simulink library "nist_library"  (R2012b)
settings: Solver=VariableStepDiscrete  StartTime=0  StopTime=1000  RelTol=1e-3
undefined symbols (not defined in the file or in its folder): A, B, C, D, sfp, xlipgetpartsetting
libraries: xbsIndex_r4 x385, xps_library x44, nist_library x4, casper_library_misc x4, casper_library_delays x1
(part 4 of 11)

== system nist_library/channelized_fir/odd_sym_tap ==
  samp_in : Inport
  sum_in : Inport  Port=2
  Constant0 : xbsIndex_r4/Constant  const=4  gui_display_data_type=Fixed-point  arith_type=Signed (2's comp)  n_bits=18  bin_pt=0  preci_type=Single  exp_width=8  frac_width=24  explicit_period=on  period=1  equ=P=C  opselect=C  inp2=PCIN>>17  opr=+  inp1=P  carry=CIN  dbl_ovrd=off  block_type=constant
  DSP48 Macro_0 : xbsIndex_r4/DSP48 Macro 2.1   dsptype=Target XtremeDSP Slice: DSP48E1  instruction_list=A * B+C  AvailableInstructions=|  show_filtered=off  pipeline_options=Expert  dspimage=|  tier_1=off  tier_2=off  tier_3=off  tier_4=off  tier_5=off  tier_6=off  dreg_1=off  dreg_2=off  dreg_3=off  areg_1=off  areg_2=off  areg_3=on  areg_4=on  breg_1=off  breg_2=off  breg_3=on  breg_4=on  mreg_5=on  concatreg_3=off  concatreg_4=off  concatreg_5=off  creg_1=off  creg_2=off  creg_3=off  creg_4=off  creg_5=on  preg_6=on  cinreg_1=off  cinreg_2=off  cinreg_3=off  cinreg_4=off  cinreg_5=off  opreg_1=off  opreg_2=off  opreg_3=off  opreg_4=off  opreg_5=off  output_properties=Full_Precision  p_width=39  p_binarywidth=0  has_acout=off  has_bcout=off  has_pcout=off  has_carryout=off  has_carrycascout=off  has_ce=off  has_d_ce=off  has_a_ce=off  has_b_ce=off  has_concat_ce=off  has_c_ce=off  has_m_ce=off  has_p_ce=off  has_sel_ce=off  has_sclr=off  has_d_sclr=off  has_a_sclr=off  has_b_sclr=off  has_concat_sclr=off  has_c_sclr=off  has_m_sclr=off  has_p_sclr=off  has_sel_sclr=off  use_dsp48=on  gui_behaviour=Sysgen  instruction1=#  ip_name=DSP48 Macro  ip_version=2.1  dsptool_ready=true  ipcore_usecache=true  ipcore_useipmodelcache=true  wrapper_available=true  port_translation_map={ 'ce' => 'en', 'sclr' => 'rst'}  ipcore_xco_need_fpga_part=true  ipcore_fpga_part=xlipgetpartsetting(gcb, {'virtex6', 'xc6vlx75t', '-3', 'ff784'})  ipcore_latency_function='has_combinational'  structural_sim=false  ipcore_verbose=false  ipcore_port_config={ 'carryin' => { 'arith' => 'ufix', 'binpt' => 0.00000000000, 'width' => 1.00000000000}, 'carrycascin' => { 'arith' => 'ufix', 'binpt' => 0.00000000000, 'width' => 1.00000000000}, 'carrycascout' => { 'arith' => 'ufix', 'binpt' => 0.00000000000, 'width' => 1.00000000000}, 'carryout' => { 'arith' => 'ufix', 'binpt' => 0.00000000000, 'width' => 1.00000000000}}  block_type=xbip_dsp48_macro_v2_1
      AvailableInstructions=|
      | '(A+D)
      | (A+D)*B
      | (A+D)*B+C
      | (A+D)*B+C+CARRYIN
      | (A+D)*B+CARRYIN
      | (A+D)*B+P
      | (A+D)*B+P+CARRYIN
      | (A+D)*B+P>>17
      | (A+D)*B+P>>17+CARRYIN
      | (A+D)*B+PCIN
      | (A+D)*B+PCIN+CARRYIN
      | (A+D)*B+PCIN>>17
      | (A+D)*B+PCIN>>17+CARRYIN
      | (A+D)*BCIN
      | (A+D)*BCIN+C
      | (A+D)*BCIN+C+CARRYIN
      | (A+D)*BCIN+CARRYIN
      | (A+D)*BCIN+P
      | (A+D)*BCIN+P+CARRYIN
      | (A+D)*BCIN+P>>17
      | (A+D)*BCIN+P>>17+CARRYIN
      | (A+D)*BCIN+PCIN
      | (A+D)*BCIN+PCIN+CARRYIN
      | (A+D)*BCIN+PCIN>>17
      | (A+D)*BCIN+PCIN>>17+CARRYIN
      | (A+D)+C
      | (A+D)+C+CARRYIN
      | (A+D)+CARRYIN
      | (A+D)+P
      | (A+D)+P+CARRYIN
      | (A+D)+P>>17
      | (A+D)+P>>17+CARRYIN
      | (A+D)+PCIN
      | (A+D)+PCIN+CARRYIN
      | (A+D)+PCIN>>17
      | (A+D)+PCIN>>17+CARRYIN
      | (ACIN+D)
      | (ACIN+D)*B
      | (ACIN+D)*B+C
      | (ACIN+D)*B+C+CARRYIN
      | (ACIN+D)*B+CARRYIN
      | (ACIN+D)*B+P
      | (ACIN+D)*B+P+CARRYIN
      | (ACIN+D)*B+P>>17
      | (ACIN+D)*B+P>>17+CARRYIN
      | (ACIN+D)*B+PCIN
      | (ACIN+D)*B+PCIN+CARRYIN
      | (ACIN+D)*B+PCIN>>17
      | (ACIN+D)*B+PCIN>>17+CARRYIN
      | (ACIN+D)*BCIN
      | (ACIN+D)*BCIN+C
      | (ACIN+D)*BCIN+C+CARRYIN
      | (ACIN+D)*BCIN+CARRYIN
      | (ACIN+D)*BCIN+P
      | (ACIN+D)*BCIN+P+CARRYIN
      | (ACIN+D)*BCIN+P>>17
      | (ACIN+D)*BCIN+P>>17+CARRYIN
      | (ACIN+D)*BCIN+PCIN
      | (ACIN+D)*BCIN+PCIN+CARRYIN
      | (ACIN+D)*BCIN+PCIN>>17
      | (ACIN+D)*BCIN+PCIN>>17+CARRYIN
      | (ACIN+D)+C
      | (ACIN+D)+C+CARRYIN
      | (ACIN+D)+CARRYIN
      | (ACIN+D)+P
      | (ACIN+D)+P+CARRYIN
      | (ACIN+D)+P>>17
      | (ACIN+D)+P>>17+CARRYIN
      | (ACIN+D)+PCIN
      | (ACIN+D)+PCIN+CARRYIN
      | (ACIN+D)+PCIN>>17
      | (ACIN+D)+PCIN>>17+CARRYIN
      | (D+A)
      | (D+A)*B
      | (D+A)*B+C
      | (D+A)*B+C+CARRYIN
      | (D+A)*B+CARRYIN
      | (D+A)*B+P
      | (D+A)*B+P+CARRYIN
      | (D+A)*B+P>>17
      | (D+A)*B+P>>17+CARRYIN
      | (D+A)*B+PCIN
      | (D+A)*B+PCIN+CARRYIN
      | (D+A)*B+PCIN>>17
      | (D+A)*B+PCIN>>17+CARRYIN
      | (D+A)*BCIN
      | (D+A)*BCIN+C
      | (D+A)*BCIN+C+CARRYIN
      | (D+A)*BCIN+CARRYIN
      | (D+A)*BCIN+P
      | (D+A)*BCIN+P+CARRYIN
      | (D+A)*BCIN+P>>17
      | (D+A)*BCIN+P>>17+CARRYIN
      | (D+A)*BCIN+PCIN
      | (D+A)*BCIN+PCIN+CARRYIN
      | (D+A)*BCIN+PCIN>>17
      | (D+A)*BCIN+PCIN>>17+CARRYIN
      | (D+A)+C
      | (D+A)+C+CARRYIN
      | (D+A)+CARRYIN
      | (D+A)+P
      | (D+A)+P+CARRYIN
      | (D+A)+P>>17
      | (D+A)+P>>17+CARRYIN
      | (D+A)+PCIN
      | (D+A)+PCIN+CARRYIN
      | (D+A)+PCIN>>17
      | (D+A)+PCIN>>17+CARRYIN
      | (D+ACIN)
      | (D+ACIN)*B
      | (D+ACIN)*B+C
      | (D+ACIN)*B+C+CARRYIN
      | (D+ACIN)*B+CARRYIN
      | (D+ACIN)*B+P
      | (D+ACIN)*B+P+CARRYIN
      | (D+ACIN)*B+P>>17
      | (D+ACIN)*B+P>>17+CARRYIN
      | (D+ACIN)*B+PCIN
      | (D+ACIN)*B+PCIN+CARRYIN
      | (D+ACIN)*B+PCIN>>17
      | (D+ACIN)*B+PCIN>>17+CARRYIN
      | (D+ACIN)*BCIN
      | (D+ACIN)*BCIN+C
      | (D+ACIN)*BCIN+C+CARRYIN
      | (D+ACIN)*BCIN+CARRYIN
      | (D+ACIN)*BCIN+P
      | (D+ACIN)*BCIN+P+CARRYIN
      | (D+ACIN)*BCIN+P>>17
      | (D+ACIN)*BCIN+P>>17+CARRYIN
      | (D+ACIN)*BCIN+PCIN
      | (D+ACIN)*BCIN+PCIN+CARRYIN
      | (D+ACIN)*BCIN+PCIN>>17
      | (D+ACIN)*BCIN+PCIN>>17+CARRYIN
      | (D+ACIN)+C
      | (D+ACIN)+C+CARRYIN
      | (D+ACIN)+CARRYIN
      | (D+ACIN)+P
      | (D+ACIN)+P+CARRYIN
      | (D+ACIN)+P>>17
      | (D+ACIN)+P>>17+CARRYIN
      | (D+ACIN)+PCIN
      | (D+ACIN)+PCIN+CARRYIN
      | (D+ACIN)+PCIN>>17
      | (D+ACIN)+PCIN>>17+CARRYIN
      | (D-A)
      | (D-A)*B
      | (D-A)*B+C
      | (D-A)*B+C+CARRYIN
      | (D-A)*B+CARRYIN
      | (D-A)*B+P
      | (D-A)*B+P+CARRYIN
      | (D-A)*B+P>>17
      | (D-A)*B+P>>17+CARRYIN
      | (D-A)*B+PCIN
      | (D-A)*B+PCIN+CARRYIN
      | (D-A)*B+PCIN>>17
      | (D-A)*B+PCIN>>17+CARRYIN
      | (D-A)*BCIN
      | (D-A)*BCIN+C
      | (D-A)*BCIN+C+CARRYIN
      | (D-A)*BCIN+CARRYIN
      | (D-A)*BCIN+P
      | (D-A)*BCIN+P+CARRYIN
      | (D-A)*BCIN+P>>17
      | (D-A)*BCIN+P>>17+CARRYIN
      | (D-A)*BCIN+PCIN
      | (D-A)*BCIN+PCIN+CARRYIN
      | (D-A)*BCIN+PCIN>>17
      | (D-A)*BCIN+PCIN>>17+CARRYIN
      | (D-A)+C
      | (D-A)+C+CARRYIN
      | (D-A)+CARRYIN
      | (D-A)+P
      | (D-A)+P+CARRYIN
      | (D-A)+P>>17
      | (D-A)+P>>17+CARRYIN
      | (D-A)+PCIN
      | (D-A)+PCIN+CARRYIN
      | (D-A)+PCIN>>17
      | (D-A)+PCIN>>17+CARRYIN
      | (D-ACIN)
      | (D-ACIN)*B
      | (D-ACIN)*B+C
      | (D-ACIN)*B+C+CARRYIN
      | (D-ACIN)*B+CARRYIN
      | (D-ACIN)*B+P
      | (D-ACIN)*B+P+CARRYIN
      | (D-ACIN)*B+P>>17
      | (D-ACIN)*B+P>>17+CARRYIN
      | (D-ACIN)*B+PCIN
      | (D-ACIN)*B+PCIN+CARRYIN
      | (D-ACIN)*B+PCIN>>17
      | (D-ACIN)*B+PCIN>>17+CARRYIN
      | (D-ACIN)*BCIN
      | (D-ACIN)*BCIN+C
      | (D-ACIN)*BCIN+C+CARRYIN
      | (D-ACIN)*BCIN+CARRYIN
      | (D-ACIN)*BCIN+P
      | (D-ACIN)*BCIN+P+CARRYIN
      | (D-ACIN)*BCIN+P>>17
      | (D-ACIN)*BCIN+P>>17+CARRYIN
      | (D-ACIN)*BCIN+PCIN
      | (D-ACIN)*BCIN+PCIN+CARRYIN
      | (D-ACIN)*BCIN+PCIN>>17
      | (D-ACIN)*BCIN+PCIN>>17+CARRYIN
      | (D-ACIN)+C
      | (D-ACIN)+C+CARRYIN
      | (D-ACIN)+CARRYIN
      | (D-ACIN)+P
      | (D-ACIN)+P+CARRYIN
      | (D-ACIN)+P>>17
      | (D-ACIN)+P>>17+CARRYIN
      | (D-ACIN)+PCIN
      | (D-ACIN)+PCIN+CARRYIN
      | (D-ACIN)+PCIN>>17
      | (D-ACIN)+PCIN>>17+CARRYIN
      | -((A+D))
      | -((A+D)*B)
      | -((A+D)*B+CARRYIN)
      | -((A+D)*BCIN)
      | -((A+D)*BCIN+CARRYIN)
      | -((A+D)+CARRYIN)
      | -((ACIN+D))
      | -((ACIN+D)*B)
      | -((ACIN+D)*B+CARRYIN)
      | -((ACIN+D)*BCIN)
      | -((ACIN+D)*BCIN+CARRYIN)
      | -((ACIN+D)+CARRYIN)
      | -((D+A))
      | -((D+A)*B)
      | -((D+A)*B+CARRYIN)
      | -((D+A)*BCIN)
      | -((D+A)*BCIN+CARRYIN)
      | -((D+A)+CARRYIN)
      | -((D+ACIN))
      | -((D+ACIN)*B)
      | -((D+ACIN)*B+CARRYIN)
      | -((D+ACIN)*BCIN)
      | -((D+ACIN)*BCIN+CARRYIN)
      | -((D+ACIN)+CARRYIN)
      | -((D-A))
      | -((D-A)*B)
      | -((D-A)*B+CARRYIN)
      | -((D-A)*BCIN)
      | -((D-A)*BCIN+CARRYIN)
      | -((D-A)+CARRYIN)
      | -((D-ACIN))
      | -((D-ACIN)*B)
      | -((D-ACIN)*B+CARRYIN)
      | -((D-ACIN)*BCIN)
      | -((D-ACIN)*BCIN+CARRYIN)
      | -((D-ACIN)+CARRYIN)
      | -(A)
      | -(A*B)
      | -(A*B+CARRYIN)
      | -(A*BCIN)
      | -(A*BCIN+CARRYIN)
      | -(A+CARRYIN)
      | -(A+D)
      | -(A+D)*B
      | -(A+D)*B-CARRYIN
      | -(A+D)*BCIN
      | -(A+D)*BCIN-CARRYIN
      | -(A+D)-CARRYIN
      | -(ACIN)
      | -(ACIN*B)
      | -(ACIN*B+CARRYIN)
      | -(ACIN*BCIN)
      | -(ACIN*BCIN+CARRYIN)
      | -(ACIN+CARRYIN)
      | -(ACIN+D)
      | -(ACIN+D)*B
      | -(ACIN+D)*B-CARRYIN
      | -(ACIN+D)*BCIN
      | -(ACIN+D)*BCIN-CARRYIN
      | -(ACIN+D)-CARRYIN
      | -(B*(A+D))
      | -(B*(A+D)+CARRYIN)
      | -(B*(ACIN+D))
      | -(B*(ACIN+D)+CARRYIN)
      | -(B*(D+A))
      | -(B*(D+A)+CARRYIN)
      | -(B*(D+ACIN))
      | -(B*(D+ACIN)+CARRYIN)
      | -(B*(D-A))
      | -(B*(D-A)+CARRYIN)
      | -(B*(D-ACIN))
      | -(B*(D-ACIN)+CARRYIN)
      | -(B*A)
      | -(B*A+CARRYIN)
      | -(B*ACIN)
      | -(B*ACIN+CARRYIN)
      | -(B*D)
      | -(B*D+CARRYIN)
      | -(BCIN*(A+D))
      | -(BCIN*(A+D)+CARRYIN)
      | -(BCIN*(ACIN+D))
      | -(BCIN*(ACIN+D)+CARRYIN)
      | -(BCIN*(D+A))
      | -(BCIN*(D+A)+CARRYIN)
      | -(BCIN*(D+ACIN))
      | -(BCIN*(D+ACIN)+CARRYIN)
      | -(BCIN*(D-A))
      | -(BCIN*(D-A)+CARRYIN)
      | -(BCIN*(D-ACIN))
      | -(BCIN*(D-ACIN)+CARRYIN)
      | -(BCIN*A)
      | -(BCIN*A+CARRYIN)
      | -(BCIN*ACIN)
      | -(BCIN*ACIN+CARRYIN)
      | -(BCIN*D)
      | -(BCIN*D+CARRYIN)
      | -(C)
      | -(C+CARRYCASCIN)
      | -(C+CARRYIN)
      | -(C+CONCAT)
      | -(C+CONCAT+CARRYCASCIN)
      | -(C+CONCAT+CARRYIN)
      | -(C+P)
      | -(C+P+CARRYCASCIN)
      | -(C+P+CARRYIN)
      | -(CARRYIN)
      | -(CONCAT)
      | -(CONCAT+C)
      | -(CONCAT+C+CARRYCASCIN)
      | -(CONCAT+C+CARRYIN)
      | -(CONCAT+CARRYCASCIN)
      | -(CONCAT+CARRYIN)
      | -(D)
      | -(D*B)
      | -(D*B+CARRYIN)
      | -(D*BCIN)
      | -(D*BCIN+CARRYIN)
      | -(D+A)
      | -(D+A)*B
      | -(D+A)*B-CARRYIN
      | -(D+A)*BCIN
      | -(D+A)*BCIN-CARRYIN
      | -(D+A)-CARRYIN
      | -(D+ACIN)
      | -(D+ACIN)*B
      | -(D+ACIN)*B-CARRYIN
      | -(D+ACIN)*BCIN
      | -(D+ACIN)*BCIN-CARRYIN
      | -(D+ACIN)-CARRYIN
      | -(D+CARRYIN)
      | -(D-A)
      | -(D-A)*B
      | -(D-A)*B-CARRYIN
      | -(D-A)*BCIN
      | -(D-A)*BCIN-CARRYIN
      | -(D-A)-CARRYIN
      | -(D-ACIN)
      | -(D-ACIN)*B
      | -(D-ACIN)*B-CARRYIN
      | -(D-ACIN)*BCIN
      | -(D-ACIN)*BCIN-CARRYIN
      | -(D-ACIN)-CARRYIN
      | -(P)
      | -(P+C)
      | -(P+C+CARRYCASCIN)
      | -(P+C+CARRYIN)
      | -(P+CARRYCASCIN)
      | -(P+CARRYIN)
      | -A
      | -A*B
      | -A*B-CARRYIN
      | -A*BCIN
      | -A*BCIN-CARRYIN
      | -A-CARRYIN
      | -ACIN
      | -ACIN*B
      | -ACIN*B-CARRYIN
      | -ACIN*BCIN
      | -ACIN*BCIN-CARRYIN
      | -ACIN-CARRYIN
      | -B*(A+D)
      | -B*(A+D)-CARRYIN
      | -B*(ACIN+D)
      | -B*(ACIN+D)-CARRYIN
      | -B*(D+A)
      | -B*(D+A)-CARRYIN
      | -B*(D+ACIN)
      | -B*(D+ACIN)-CARRYIN
      | -B*(D-A)
      | -B*(D-A)-CARRYIN
      | -B*(D-ACIN)
      | -B*(D-ACIN)-CARRYIN
      | -B*A
      | -B*A-CARRYIN
      | -B*ACIN
      | -B*ACIN-CARRYIN
      | -B*D
      | -B*D-CARRYIN
      | -BCIN*(A+D)
      | -BCIN*(A+D)-CARRYIN
      | -BCIN*(ACIN+D)
      | -BCIN*(ACIN+D)-CARRYIN
      | -BCIN*(D+A)
      | -BCIN*(D+A)-CARRYIN
      | -BCIN*(D+ACIN)
      | -BCIN*(D+ACIN)-CARRYIN
      | -BCIN*(D-A)
      | -BCIN*(D-A)-CARRYIN
      | -BCIN*(D-ACIN)
      | -BCIN*(D-ACIN)-CARRYIN
      | -BCIN*A
      | -BCIN*A-CARRYIN
      | -BCIN*ACIN
      | -BCIN*ACIN-CARRYIN
      | -BCIN*D
      | -BCIN*D-CARRYIN
      | -C
      | -C-CARRYCASCIN
      | -C-CARRYIN
      | -C-CONCAT
      | -C-CONCAT-CARRYCASCIN
      | -C-CONCAT-CARRYIN
      | -C-P
      | -C-P-CARRYCASCIN
      | -C-P-CARRYIN
      | -CARRYIN
      | -CONCAT
      | -CONCAT-C
      | -CONCAT-C-CARRYCASCIN
      | -CONCAT-C-CARRYIN
      | -CONCAT-CARRYCASCIN
      | -CONCAT-CARRYIN
      | -D
      | -D*B
      | -D*B-CARRYIN
      | -D*BCIN
      | -D*BCIN-CARRYIN
      | -D-CARRYIN
      | -P
      | -P-C
      | -P-C-CARRYCASCIN
      | -P-C-CARRYIN
      | -P-CARRYCASCIN
      | -P-CARRYIN
      | 0
      | A
      | A*B
      | A*B+C
      | A*B+C+CARRYIN
      | A*B+CARRYIN
      | A*B+P
      | A*B+P+CARRYIN
      | A*B+P>>17
      | A*B+P>>17+CARRYIN
      | A*B+PCIN
      | A*B+PCIN+CARRYIN
      | A*B+PCIN>>17
      | A*B+PCIN>>17+CARRYIN
      | A*BCIN
      | A*BCIN+C
      | A*BCIN+C+CARRYIN
      | A*BCIN+CARRYIN
      | A*BCIN+P
      | A*BCIN+P+CARRYIN
      | A*BCIN+P>>17
      | A*BCIN+P>>17+CARRYIN
      | A*BCIN+PCIN
      | A*BCIN+PCIN+CARRYIN
      | A*BCIN+PCIN>>17
      | A*BCIN+PCIN>>17+CARRYIN
      | A+C
      | A+C+CARRYIN
      | A+CARRYIN
      | A+P
      | A+P+CARRYIN
      | A+P>>17
      | A+P>>17+CARRYIN
      | A+PCIN
      | A+PCIN+CARRYIN
      | A+PCIN>>17
      | A+PCIN>>17+CARRYIN
      | ACIN
      | ACIN*B
      | ACIN*B+C
      | ACIN*B+C+CARRYIN
      | ACIN*B+CARRYIN
      | ACIN*B+P
      | ACIN*B+P+CARRYIN
      | ACIN*B+P>>17
      | ACIN*B+P>>17+CARRYIN
      | ACIN*B+PCIN
      | ACIN*B+PCIN+CARRYIN
      | ACIN*B+PCIN>>17
      | ACIN*B+PCIN>>17+CARRYIN
      | ACIN*BCIN
      | ACIN*BCIN+C
      | ACIN*BCIN+C+CARRYIN
      | ACIN*BCIN+CARRYIN
      | ACIN*BCIN+P
      | ACIN*BCIN+P+CARRYIN
      | ACIN*BCIN+P>>17
      | ACIN*BCIN+P>>17+CARRYIN
      | ACIN*BCIN+PCIN
      | ACIN*BCIN+PCIN+CARRYIN
      | ACIN*BCIN+PCIN>>17
      | ACIN*BCIN+PCIN>>17+CARRYIN
      | ACIN+C
      | ACIN+C+CARRYIN
      | ACIN+CARRYIN
      | ACIN+P
      | ACIN+P+CARRYIN
      | ACIN+P>>17
      | ACIN+P>>17+CARRYIN
      | ACIN+PCIN
      | ACIN+PCIN+CARRYIN
      | ACIN+PCIN>>17
      | ACIN+PCIN>>17+CARRYIN
      | B*(A+D)
      | B*(A+D)+C
      | B*(A+D)+C+CARRYIN
      | B*(A+D)+CARRYIN
      | B*(A+D)+P
      | B*(A+D)+P+CARRYIN
      | B*(A+D)+P>>17
      | B*(A+D)+P>>17+CARRYIN
      | B*(A+D)+PCIN
      | B*(A+D)+PCIN+CARRYIN
      | B*(A+D)+PCIN>>17
      | B*(A+D)+PCIN>>17+CARRYIN
      | B*(ACIN+D)
      | B*(ACIN+D)+C
      | B*(ACIN+D)+C+CARRYIN
      | B*(ACIN+D)+CARRYIN
      | B*(ACIN+D)+P
      | B*(ACIN+D)+P+CARRYIN
      | B*(ACIN+D)+P>>17
      | B*(ACIN+D)+P>>17+CARRYIN
      | B*(ACIN+D)+PCIN
      | B*(ACIN+D)+PCIN+CARRYIN
      | B*(ACIN+D)+PCIN>>17
      | B*(ACIN+D)+PCIN>>17+CARRYIN
      | B*(D+A)
      | B*(D+A)+C
      | B*(D+A)+C+CARRYIN
      | B*(D+A)+CARRYIN
      | B*(D+A)+P
      | B*(D+A)+P+CARRYIN
      | B*(D+A)+P>>17
      | B*(D+A)+P>>17+CARRYIN
      | B*(D+A)+PCIN
      | B*(D+A)+PCIN+CARRYIN
      | B*(D+A)+PCIN>>17
      | B*(D+A)+PCIN>>17+CARRYIN
      | B*(D+ACIN)
      | B*(D+ACIN)+C
      | B*(D+ACIN)+C+CARRYIN
      | B*(D+ACIN)+CARRYIN
      | B*(D+ACIN)+P
      | B*(D+ACIN)+P+CARRYIN
      | B*(D+ACIN)+P>>17
      | B*(D+ACIN)+P>>17+CARRYIN
      | B*(D+ACIN)+PCIN
      | B*(D+ACIN)+PCIN+CARRYIN
      | B*(D+ACIN)+PCIN>>17
      | B*(D+ACIN)+PCIN>>17+CARRYIN
      | B*(D-A)
      | B*(D-A)+C
      | B*(D-A)+C+CARRYIN
      | B*(D-A)+CARRYIN
      | B*(D-A)+P
      | B*(D-A)+P+CARRYIN
      | B*(D-A)+P>>17
      | B*(D-A)+P>>17+CARRYIN
      | B*(D-A)+PCIN
      | B*(D-A)+PCIN+CARRYIN
      | B*(D-A)+PCIN>>17
      | B*(D-A)+PCIN>>17+CARRYIN
      | B*(D-ACIN)
      | B*(D-ACIN)+C
      | B*(D-ACIN)+C+CARRYIN
      | B*(D-ACIN)+CARRYIN
      | B*(D-ACIN)+P
      | B*(D-ACIN)+P+CARRYIN
      | B*(D-ACIN)+P>>17
      | B*(D-ACIN)+P>>17+CARRYIN
      | B*(D-ACIN)+PCIN
      | B*(D-ACIN)+PCIN+CARRYIN
      | B*(D-ACIN)+PCIN>>17
      | B*(D-ACIN)+PCIN>>17+CARRYIN
      | B*A
      | B*A+C
      | B*A+C+CARRYIN
      | B*A+CARRYIN
      | B*A+P
      | B*A+P+CARRYIN
      | B*A+P>>17
      | B*A+P>>17+CARRYIN
      | B*A+PCIN
      | B*A+PCIN+CARRYIN
      | B*A+PCIN>>17
      | B*A+PCIN>>17+CARRYIN
      | B*ACIN
      | B*ACIN+C
      | B*ACIN+C+CARRYIN
      | B*ACIN+CARRYIN
      | B*ACIN+P
      | B*ACIN+P+CARRYIN
      | B*ACIN+P>>17
      | B*ACIN+P>>17+CARRYIN
      | B*ACIN+PCIN
      | B*ACIN+PCIN+CARRYIN
      | B*ACIN+PCIN>>17
      | B*ACIN+PCIN>>17+CARRYIN
      | B*D
      | B*D+C
      | B*D+C+CARRYIN
      | B*D+CARRYIN
      | B*D+P
      | B*D+P+CARRYIN
      | B*D+P>>17
      | B*D+P>>17+CARRYIN
      | B*D+PCIN
      | B*D+PCIN+CARRYIN
      | B*D+PCIN>>17
      | B*D+PCIN>>17+CARRYIN
      | BCIN*(A+D)
      | BCIN*(A+D)+C
      | BCIN*(A+D)+C+CARRYIN
      | BCIN*(A+D)+CARRYIN
      | BCIN*(A+D)+P
      | BCIN*(A+D)+P+CARRYIN
      | BCIN*(A+D)+P>>17
      | BCIN*(A+D)+P>>17+CARRYIN
      | BCIN*(A+D)+PCIN
      | BCIN*(A+D)+PCIN+CARRYIN
      | BCIN*(A+D)+PCIN>>17
      | BCIN*(A+D)+PCIN>>17+CARRYIN
      | BCIN*(ACIN+D)
      | BCIN*(ACIN+D)+C
      | BCIN*(ACIN+D)+C+CARRYIN
      | BCIN*(ACIN+D)+CARRYIN
      | BCIN*(ACIN+D)+P
      | BCIN*(ACIN+D)+P+CARRYIN
      | BCIN*(ACIN+D)+P>>17
      | BCIN*(ACIN+D)+P>>17+CARRYIN
      | BCIN*(ACIN+D)+PCIN
      | BCIN*(ACIN+D)+PCIN+CARRYIN
      | BCIN*(ACIN+D)+PCIN>>17
      | BCIN*(ACIN+D)+PCIN>>17+CARRYIN
      | BCIN*(D+A)
      | BCIN*(D+A)+C
      | BCIN*(D+A)+C+CARRYIN
      | BCIN*(D+A)+CARRYIN
      | BCIN*(D+A)+P
      | BCIN*(D+A)+P+CARRYIN
      | BCIN*(D+A)+P>>17
      | BCIN*(D+A)+P>>17+CARRYIN
      | BCIN*(D+A)+PCIN
      | BCIN*(D+A)+PCIN+CARRYIN
      | BCIN*(D+A)+PCIN>>17
      | BCIN*(D+A)+PCIN>>17+CARRYIN
      | BCIN*(D+ACIN)
      | BCIN*(D+ACIN)+C
      | BCIN*(D+ACIN)+C+CARRYIN
      | BCIN*(D+ACIN)+CARRYIN
      | BCIN*(D+ACIN)+P
      | BCIN*(D+ACIN)+P+CARRYIN
      | BCIN*(D+ACIN)+P>>17
      | BCIN*(D+ACIN)+P>>17+CARRYIN
      | BCIN*(D+ACIN)+PCIN
      | BCIN*(D+ACIN)+PCIN+CARRYIN
      | BCIN*(D+ACIN)+PCIN>>17
      | BCIN*(D+ACIN)+PCIN>>17+CARRYIN
      | BCIN*(D-A)
      | BCIN*(D-A)+C
      | BCIN*(D-A)+C+CARRYIN
      | BCIN*(D-A)+CARRYIN
      | BCIN*(D-A)+P
      | BCIN*(D-A)+P+CARRYIN
      | BCIN*(D-A)+P>>17
      | BCIN*(D-A)+P>>17+CARRYIN
      | BCIN*(D-A)+PCIN
      | BCIN*(D-A)+PCIN+CARRYIN
      | BCIN*(D-A)+PCIN>>17
      | BCIN*(D-A)+PCIN>>17+CARRYIN
      | BCIN*(D-ACIN)
      | BCIN*(D-ACIN)+C
      | BCIN*(D-ACIN)+C+CARRYIN
      | BCIN*(D-ACIN)+CARRYIN
      | BCIN*(D-ACIN)+P
      | BCIN*(D-ACIN)+P+CARRYIN
      | BCIN*(D-ACIN)+P>>17
      | BCIN*(D-ACIN)+P>>17+CARRYIN
      | BCIN*(D-ACIN)+PCIN
      | BCIN*(D-ACIN)+PCIN+CARRYIN
      | BCIN*(D-ACIN)+PCIN>>17
      | BCIN*(D-ACIN)+PCIN>>17+CARRYIN
      | BCIN*A
      | BCIN*A+C
      | BCIN*A+C+CARRYIN
      | BCIN*A+CARRYIN
      | BCIN*A+P
      | BCIN*A+P+CARRYIN
      | BCIN*A+P>>17
      | BCIN*A+P>>17+CARRYIN
      | BCIN*A+PCIN
      | BCIN*A+PCIN+CARRYIN
      | BCIN*A+PCIN>>17
      | BCIN*A+PCIN>>17+CARRYIN
      | BCIN*ACIN
      | BCIN*ACIN+C
      | BCIN*ACIN+C+CARRYIN
      | BCIN*ACIN+CARRYIN
      | BCIN*ACIN+P
      | BCIN*ACIN+P+CARRYIN
      | BCIN*ACIN+P>>17
      | BCIN*ACIN+P>>17+CARRYIN
      | BCIN*ACIN+PCIN
      | BCIN*ACIN+PCIN+CARRYIN
      | BCIN*ACIN+PCIN>>17
      | BCIN*ACIN+PCIN>>17+CARRYIN
      | BCIN*D
      | BCIN*D+C
      | BCIN*D+C+CARRYIN
      | BCIN*D+CARRYIN
      | BCIN*D+P
      | BCIN*D+P+CARRYIN
      | BCIN*D+P>>17
      | BCIN*D+P>>17+CARRYIN
      | BCIN*D+PCIN
      | BCIN*D+PCIN+CARRYIN
      | BCIN*D+PCIN>>17
      | BCIN*D+PCIN>>17+CARRYIN
      | C
      | C+(A+D)
      | C+(A+D)*B
      | C+(A+D)*B+CARRYIN
      | C+(A+D)*BCIN
      | C+(A+D)*BCIN+CARRYIN
      | C+(A+D)+CARRYIN
      | C+(ACIN+D)
      | C+(ACIN+D)*B
      | C+(ACIN+D)*B+CARRYIN
      | C+(ACIN+D)*BCIN
      | C+(ACIN+D)*BCIN+CARRYIN
      | C+(ACIN+D)+CARRYIN
      | C+(D+A)
      | C+(D+A)*B
      | C+(D+A)*B+CARRYIN
      | C+(D+A)*BCIN
      | C+(D+A)*BCIN+CARRYIN
      | C+(D+A)+CARRYIN
      | C+(D+ACIN)
      | C+(D+ACIN)*B
      | C+(D+ACIN)*B+CARRYIN
      | C+(D+ACIN)*BCIN
      | C+(D+ACIN)*BCIN+CARRYIN
      | C+(D+ACIN)+CARRYIN
      | C+(D-A)
      | C+(D-A)*B
      | C+(D-A)*B+CARRYIN
      | C+(D-A)*BCIN
      | C+(D-A)*BCIN+CARRYIN
      | C+(D-A)+CARRYIN
      | C+(D-ACIN)
      | C+(D-ACIN)*B
      | C+(D-ACIN)*B+CARRYIN
      | C+(D-ACIN)*BCIN
      | C+(D-ACIN)*BCIN+CARRYIN
      | C+(D-ACIN)+CARRYIN
      | C+A
      | C+A*B
      | C+A*B+CARRYIN
      | C+A*BCIN
      | C+A*BCIN+CARRYIN
      | C+A+CARRYIN
      | C+ACIN
      | C+ACIN*B
      | C+ACIN*B+CARRYIN
      | C+ACIN*BCIN
      | C+ACIN*BCIN+CARRYIN
      | C+ACIN+CARRYIN
      | C+B*(A+D)
      | C+B*(A+D)+CARRYIN
      | C+B*(ACIN+D)
      | C+B*(ACIN+D)+CARRYIN
      | C+B*(D+A)
      | C+B*(D+A)+CARRYIN
      | C+B*(D+ACIN)
      | C+B*(D+ACIN)+CARRYIN
      | C+B*(D-A)
      | C+B*(D-A)+CARRYIN
      | C+B*(D-ACIN)
      | C+B*(D-ACIN)+CARRYIN
      | C+B*A
      | C+B*A+CARRYIN
      | C+B*ACIN
      | C+B*ACIN+CARRYIN
      | C+B*D
      | C+B*D+CARRYIN
      | C+BCIN*(A+D)
      | C+BCIN*(A+D)+CARRYIN
      | C+BCIN*(ACIN+D)
      | C+BCIN*(ACIN+D)+CARRYIN
      | C+BCIN*(D+A)
      | C+BCIN*(D+A)+CARRYIN
      | C+BCIN*(D+ACIN)
      | C+BCIN*(D+ACIN)+CARRYIN
      | C+BCIN*(D-A)
      | C+BCIN*(D-A)+CARRYIN
      | C+BCIN*(D-ACIN)
      | C+BCIN*(D-ACIN)+CARRYIN
      | C+BCIN*A
      | C+BCIN*A+CARRYIN
      | C+BCIN*ACIN
      | C+BCIN*ACIN+CARRYIN
      | C+BCIN*D
      | C+BCIN*D+CARRYIN
      | C+C
      | C+C+CARRYCASCIN
      | C+C+CARRYIN
      | C+C+CONCAT
      | C+C+CONCAT+CARRYIN
      | C+C+P
      | C+C+P+CARRYIN
      | C+CARRYCASCIN
      | C+CARRYIN
      | C+CONCAT
      | C+CONCAT+C
      | C+CONCAT+C+CARRYIN
      | C+CONCAT+CARRYCASCIN
      | C+CONCAT+CARRYIN
      | C+CONCAT+P
      | C+CONCAT+P+CARRYIN
      | C+CONCAT+P>>17
      | C+CONCAT+P>>17+CARRYIN
      | C+CONCAT+PCIN
      | C+CONCAT+PCIN+CARRYIN
      | C+CONCAT+PCIN>>17
      | C+CONCAT+PCIN>>17+CARRYIN
      | C+D
      | C+D*B
      | C+D*B+CARRYIN
      | C+D*BCIN
      | C+D*BCIN+CARRYIN
      | C+D+CARRYIN
      | C+P
      | C+P+C
      | C+P+C+CARRYIN
      | C+P+CARRYCASCIN
      | C+P+CARRYIN
      | C+P+CONCAT
      | C+P+CONCAT+CARRYIN
      | C+P+P
      | C+P+P+CARRYIN
      | C+P+P>>17
      | C+P+P>>17+CARRYIN
      | C+P+PCIN
      | C+P+PCIN+CARRYIN
      | C+P+PCIN>>17
      | C+P+PCIN>>17+CARRYIN
      | C+P>>17
      | C+P>>17+CARRYIN
      | C+P>>17+CONCAT
      | C+P>>17+CONCAT+CARRYIN
      | C+P>>17+P
      | C+P>>17+P+CARRYIN
      | C+PCIN
      | C+PCIN+CARRYIN
      | C+PCIN+CONCAT
      | C+PCIN+CONCAT+CARRYIN
      | C+PCIN+P
      | C+PCIN+P+CARRYIN
      | C+PCIN>>17
      | C+PCIN>>17+CARRYIN
      | C+PCIN>>17+CONCAT
      | C+PCIN>>17+CONCAT+CARRYIN
      | C+PCIN>>17+P
      | C+PCIN>>17+P+CARRYIN
      | C-((A+D))
      | C-((A+D)*B)
      | C-((A+D)*B+CARRYIN)
      | C-((A+D)*BCIN)
      | C-((A+D)*BCIN+CARRYIN)
      | C-((A+D)+CARRYIN)
      | C-((ACIN+D))
      | C-((ACIN+D)*B)
      | C-((ACIN+D)*B+CARRYIN)
      | C-((ACIN+D)*BCIN)
      | C-((ACIN+D)*BCIN+CARRYIN)
      | C-((ACIN+D)+CARRYIN)
      | C-((D+A))
      | C-((D+A)*B)
      | C-((D+A)*B+CARRYIN)
      | C-((D+A)*BCIN)
      | C-((D+A)*BCIN+CARRYIN)
      | C-((D+A)+CARRYIN)
      | C-((D+ACIN))
      | C-((D+ACIN)*B)
      | C-((D+ACIN)*B+CARRYIN)
      | C-((D+ACIN)*BCIN)
      | C-((D+ACIN)*BCIN+CARRYIN)
      | C-((D+ACIN)+CARRYIN)
      | C-((D-A))
      | C-((D-A)*B)
      | C-((D-A)*B+CARRYIN)
      | C-((D-A)*BCIN)
      | C-((D-A)*BCIN+CARRYIN)
      | C-((D-A)+CARRYIN)
      | C-((D-ACIN))
      | C-((D-ACIN)*B)
      | C-((D-ACIN)*B+CARRYIN)
      | C-((D-ACIN)*BCIN)
      | C-((D-ACIN)*BCIN+CARRYIN)
      | C-((D-ACIN)+CARRYIN)
      | C-(A)
      | C-(A*B)
      | C-(A*B+CARRYIN)
      | C-(A*BCIN)
      | C-(A*BCIN+CARRYIN)
      | C-(A+CARRYIN)
      | C-(A+D)
      | C-(A+D)*B
      | C-(A+D)*B-CARRYIN
      | C-(A+D)*BCIN
      | C-(A+D)*BCIN-CARRYIN
      | C-(A+D)-CARRYIN
      | C-(ACIN)
      | C-(ACIN*B)
      | C-(ACIN*B+CARRYIN)
      | C-(ACIN*BCIN)
      | C-(ACIN*BCIN+CARRYIN)
      | C-(ACIN+CARRYIN)
      | C-(ACIN+D)
      | C-(ACIN+D)*B
      | C-(ACIN+D)*B-CARRYIN
      | C-(ACIN+D)*BCIN
      | C-(ACIN+D)*BCIN-CARRYIN
      | C-(ACIN+D)-CARRYIN
      | C-(B*(A+D))
      | C-(B*(A+D)+CARRYIN)
      | C-(B*(ACIN+D))
      | C-(B*(ACIN+D)+CARRYIN)
      | C-(B*(D+A))
      | C-(B*(D+A)+CARRYIN)
      | C-(B*(D+ACIN))
      | C-(B*(D+ACIN)+CARRYIN)
      | C-(B*(D-A))
      | C-(B*(D-A)+CARRYIN)
      | C-(B*(D-ACIN))
      | C-(B*(D-ACIN)+CARRYIN)
      | C-(B*A)
      | C-(B*A+CARRYIN)
      | C-(B*ACIN)
      | C-(B*ACIN+CARRYIN)
      | C-(B*D)
      | C-(B*D+CARRYIN)
      | C-(BCIN*(A+D))
      | C-(BCIN*(A+D)+CARRYIN)
      | C-(BCIN*(ACIN+D))
      | C-(BCIN*(ACIN+D)+CARRYIN)
      | C-(BCIN*(D+A))
      | C-(BCIN*(D+A)+CARRYIN)
      | C-(BCIN*(D+ACIN))
      | C-(BCIN*(D+ACIN)+CARRYIN)
      | C-(BCIN*(D-A))
      | C-(BCIN*(D-A)+CARRYIN)
      | C-(BCIN*(D-ACIN))
      | C-(BCIN*(D-ACIN)+CARRYIN)
      | C-(BCIN*A)
      | C-(BCIN*A+CARRYIN)
      | C-(BCIN*ACIN)
      | C-(BCIN*ACIN+CARRYIN)
      | C-(BCIN*D)
      | C-(BCIN*D+CARRYIN)
      | C-(C)
      | C-(C+CARRYCASCIN)
      | C-(C+CARRYIN)
      | C-(C+CONCAT)
      | C-(C+CONCAT+CARRYIN)
      | C-(C+P)
      | C-(C+P+CARRYIN)
      | C-(CARRYCASCIN)
      | C-(CARRYIN)
      | C-(CONCAT)
      | C-(CONCAT+C)
      | C-(CONCAT+C+CARRYIN)
      | C-(CONCAT+CARRYCASCIN)
      | C-(CONCAT+CARRYIN)
      | C-(D)
      | C-(D*B)
      | C-(D*B+CARRYIN)
      | C-(D*BCIN)
      | C-(D*BCIN+CARRYIN)
      | C-(D+A)
      | C-(D+A)*B
      | C-(D+A)*B-CARRYIN
      | C-(D+A)*BCIN
      | C-(D+A)*BCIN-CARRYIN
      | C-(D+A)-CARRYIN
      | C-(D+ACIN)
      | C-(D+ACIN)*B
      | C-(D+ACIN)*B-CARRYIN
      | C-(D+ACIN)*BCIN
      | C-(D+ACIN)*BCIN-CARRYIN
      | C-(D+ACIN)-CARRYIN
      | C-(D+CARRYIN)
      | C-(D-A)
      | C-(D-A)*B
      | C-(D-A)*B-CARRYIN
      | C-(D-A)*BCIN
      | C-(D-A)*BCIN-CARRYIN
      | C-(D-A)-CARRYIN
      | C-(D-ACIN)
      | C-(D-ACIN)*B
      | C-(D-ACIN)*B-CARRYIN
      | C-(D-ACIN)*BCIN
      | C-(D-ACIN)*BCIN-CARRYIN
      | C-(D-ACIN)-CARRYIN
      | C-(P)
      | C-(P+C)
      | C-(P+C+CARRYIN)
      | C-(P+CARRYCASCIN)
      | C-(P+CARRYIN)
      | C-A
      | C-A*B
      | C-A*B-CARRYIN
      | C-A*BCIN
      | C-A*BCIN-CARRYIN
      | C-A-CARRYIN
      | C-ACIN
      | C-ACIN*B
      | C-ACIN*B-CARRYIN
      | C-ACIN*BCIN
      | C-ACIN*BCIN-CARRYIN
      | C-ACIN-CARRYIN
      | C-B*(A+D)
      | C-B*(A+D)-CARRYIN
      | C-B*(ACIN+D)
      | C-B*(ACIN+D)-CARRYIN
      | C-B*(D+A)
      | C-B*(D+A)-CARRYIN
      | C-B*(D+ACIN)
      | C-B*(D+ACIN)-CARRYIN
      | C-B*(D-A)
      | C-B*(D-A)-CARRYIN
      | C-B*(D-ACIN)
      | C-B*(D-ACIN)-CARRYIN
      | C-B*A
      | C-B*A-CARRYIN
      | C-B*ACIN
      | C-B*ACIN-CARRYIN
      | C-B*D
      | C-B*D-CARRYIN
      | C-BCIN*(A+D)
      | C-BCIN*(A+D)-CARRYIN
      | C-BCIN*(ACIN+D)
      | C-BCIN*(ACIN+D)-CARRYIN
      | C-BCIN*(D+A)
      | C-BCIN*(D+A)-CARRYIN
      | C-BCIN*(D+ACIN)
      | C-BCIN*(D+ACIN)-CARRYIN
      | C-BCIN*(D-A)
      | C-BCIN*(D-A)-CARRYIN
      | C-BCIN*(D-ACIN)
      | C-BCIN*(D-ACIN)-CARRYIN
      | C-BCIN*A
      | C-BCIN*A-CARRYIN
      | C-BCIN*ACIN
      | C-BCIN*ACIN-CARRYIN
      | C-BCIN*D
      | C-BCIN*D-CARRYIN
      | C-C
      | C-C-CARRYCASCIN
      | C-C-CARRYIN
      | C-C-CONCAT
      | C-C-CONCAT-CARRYIN
      | C-C-P
      | C-C-P-CARRYIN
      | C-CARRYCASCIN
      | C-CARRYIN
      | C-CONCAT
      | C-CONCAT-C
      | C-CONCAT-C-CARRYIN
      | C-CONCAT-CARRYCASCIN
      | C-CONCAT-CARRYIN
      | C-D
      | C-D*B
      | C-D*B-CARRYIN
      | C-D*BCIN
      | C-D*BCIN-CARRYIN
      | C-D-CARRYIN
      | C-P
      | C-P-C
      | C-P-C-CARRYIN
      | C-P-CARRYCASCIN
      | C-P-CARRYIN
      | CARRYIN
      | CONCAT
      | CONCAT+C
      | CONCAT+C+C
      | CONCAT+C+C+CARRYIN
      | CONCAT+C+CARRYCASCIN
      | CONCAT+C+CARRYIN
      | CONCAT+C+P
      | CONCAT+C+P+CARRYIN
      | CONCAT+C+P>>17
      | CONCAT+C+P>>17+CARRYIN
      | CONCAT+C+PCIN
      | CONCAT+C+PCIN+CARRYIN
      | CONCAT+C+PCIN>>17
      | CONCAT+C+PCIN>>17+CARRYIN
      | CONCAT+CARRYCASCIN
      | CONCAT+CARRYIN
      | CONCAT+P
      | CONCAT+P+C
      | CONCAT+P+C+CARRYIN
      | CONCAT+P+CARRYCASCIN
      | CONCAT+P+CARRYIN
      | CONCAT+P>>17
      | CONCAT+P>>17+C
      | CONCAT+P>>17+C+CARRYIN
      | CONCAT+P>>17+CARRYIN
      | CONCAT+PCIN
      | CONCAT+PCIN+C
      | CONCAT+PCIN+C+CARRYIN
      | CONCAT+PCIN+CARRYIN
      | CONCAT+PCIN>>17
      | CONCAT+PCIN>>17+C
      | CONCAT+PCIN>>17+C+CARRYIN
      | CONCAT+PCIN>>17+CARRYIN
      | D
      | D*B
      | D*B+C
      | D*B+C+CARRYIN
      | D*B+CARRYIN
      | D*B+P
      | D*B+P+CARRYIN
      | D*B+P>>17
      | D*B+P>>17+CARRYIN
      | D*B+PCIN
      | D*B+PCIN+CARRYIN
      | D*B+PCIN>>17
      | D*B+PCIN>>17+CARRYIN
      | D*BCIN
      | D*BCIN+C
      | D*BCIN+C+CARRYIN
      | D*BCIN+CARRYIN
      | D*BCIN+P
      | D*BCIN+P+CARRYIN
      | D*BCIN+P>>17
      | D*BCIN+P>>17+CARRYIN
      | D*BCIN+PCIN
      | D*BCIN+PCIN+CARRYIN
      | D*BCIN+PCIN>>17
      | D*BCIN+PCIN>>17+CARRYIN
      | D+C
      | D+C+CARRYIN
      | D+CARRYIN
      | D+P
      | D+P+CARRYIN
      | D+P>>17
      | D+P>>17+CARRYIN
      | D+PCIN
      | D+PCIN+CARRYIN
      | D+PCIN>>17
      | D+PCIN>>17+CARRYIN
      | P
      | P+(A+D)
      | P+(A+D)*B
      | P+(A+D)*B+CARRYIN
      | P+(A+D)*BCIN
      | P+(A+D)*BCIN+CARRYIN
      | P+(A+D)+CARRYIN
      | P+(ACIN+D)
      | P+(ACIN+D)*B
      | P+(ACIN+D)*B+CARRYIN
      | P+(ACIN+D)*BCIN
      | P+(ACIN+D)*BCIN+CARRYIN
      | P+(ACIN+D)+CARRYIN
      | P+(D+A)
      | P+(D+A)*B
      | P+(D+A)*B+CARRYIN
      | P+(D+A)*BCIN
      | P+(D+A)*BCIN+CARRYIN
      | P+(D+A)+CARRYIN
      | P+(D+ACIN)
      | P+(D+ACIN)*B
      | P+(D+ACIN)*B+CARRYIN
      | P+(D+ACIN)*BCIN
      | P+(D+ACIN)*BCIN+CARRYIN
      | P+(D+ACIN)+CARRYIN
      | P+(D-A)
      | P+(D-A)*B
      | P+(D-A)*B+CARRYIN
      | P+(D-A)*BCIN
      | P+(D-A)*BCIN+CARRYIN
      | P+(D-A)+CARRYIN
      | P+(D-ACIN)
      | P+(D-ACIN)*B
      | P+(D-ACIN)*B+CARRYIN
      | P+(D-ACIN)*BCIN
      | P+(D-ACIN)*BCIN+CARRYIN
      | P+(D-ACIN)+CARRYIN
      | P+A
      | P+A*B
      | P+A*B+CARRYIN
      | P+A*BCIN
      | P+A*BCIN+CARRYIN
      | P+A+CARRYIN
      | P+ACIN
      | P+ACIN*B
      | P+ACIN*B+CARRYIN
      | P+ACIN*BCIN
      | P+ACIN*BCIN+CARRYIN
      | P+ACIN+CARRYIN
      | P+B*(A+D)
      | P+B*(A+D)+CARRYIN
      | P+B*(ACIN+D)
      | P+B*(ACIN+D)+CARRYIN
      | P+B*(D+A)
      | P+B*(D+A)+CARRYIN
      | P+B*(D+ACIN)
      | P+B*(D+ACIN)+CARRYIN
      | P+B*(D-A)
      | P+B*(D-A)+CARRYIN
      | P+B*(D-ACIN)
      | P+B*(D-ACIN)+CARRYIN
      | P+B*A
      | P+B*A+CARRYIN
      | P+B*ACIN
      | P+B*ACIN+CARRYIN
      | P+B*D
      | P+B*D+CARRYIN
      | P+BCIN*(A+D)
      | P+BCIN*(A+D)+CARRYIN
      | P+BCIN*(ACIN+D)
      | P+BCIN*(ACIN+D)+CARRYIN
      | P+BCIN*(D+A)
      | P+BCIN*(D+A)+CARRYIN
      | P+BCIN*(D+ACIN)
      | P+BCIN*(D+ACIN)+CARRYIN
      | P+BCIN*(D-A)
      | P+BCIN*(D-A)+CARRYIN
      | P+BCIN*(D-ACIN)
      | P+BCIN*(D-ACIN)+CARRYIN
      | P+BCIN*A
      | P+BCIN*A+CARRYIN
      | P+BCIN*ACIN
      | P+BCIN*ACIN+CARRYIN
      | P+BCIN*D
      | P+BCIN*D+CARRYIN
      | P+C
      | P+C+C
      | P+C+C+CARRYIN
      | P+C+CARRYCASCIN
      | P+C+CARRYIN
      | P+C+CONCAT
      | P+C+CONCAT+CARRYIN
      | P+C+P
      | P+C+P+CARRYIN
      | P+C+P>>17
      | P+C+P>>17+CARRYIN
      | P+C+PCIN
      | P+C+PCIN+CARRYIN
      | P+C+PCIN>>17
      | P+C+PCIN>>17+CARRYIN
      | P+CARRYCASCIN
      | P+CARRYIN
      | P+CONCAT
      | P+CONCAT+C
      | P+CONCAT+C+CARRYIN
      | P+CONCAT+CARRYCASCIN
      | P+CONCAT+CARRYIN
      | P+D
      | P+D*B
      | P+D*B+CARRYIN
      | P+D*BCIN
      | P+D*BCIN+CARRYIN
      | P+D+CARRYIN
      | P+P
      | P+P+C
      | P+P+C+CARRYIN
      | P+P+CARRYCASCIN
      | P+P+CARRYIN
      | P+P>>17
      | P+P>>17+C
      | P+P>>17+C+CARRYIN
      | P+P>>17+CARRYIN
      | P+PCIN
      | P+PCIN+C
      | P+PCIN+C+CARRYIN
      | P+PCIN+CARRYIN
      | P+PCIN>>17
      | P+PCIN>>17+C
      | P+PCIN>>17+C+CARRYIN
      | P+PCIN>>17+CARRYIN
      | P-((A+D))
      | P-((A+D)*B)
      | P-((A+D)*B+CARRYIN)
      | P-((A+D)*BCIN)
      | P-((A+D)*BCIN+CARRYIN)
      | P-((A+D)+CARRYIN)
      | P-((ACIN+D))
      | P-((ACIN+D)*B)
      | P-((ACIN+D)*B+CARRYIN)
      | P-((ACIN+D)*BCIN)
      | P-((ACIN+D)*BCIN+CARRYIN)
      | P-((ACIN+D)+CARRYIN)
      | P-((D+A))
      | P-((D+A)*B)
      | P-((D+A)*B+CARRYIN)
      | P-((D+A)*BCIN)
      | P-((D+A)*BCIN+CARRYIN)
      | P-((D+A)+CARRYIN)
      | P-((D+ACIN))
      | P-((D+ACIN)*B)
      | P-((D+ACIN)*B+CARRYIN)
      | P-((D+ACIN)*BCIN)
      | P-((D+ACIN)*BCIN+CARRYIN)
      | P-((D+ACIN)+CARRYIN)
      | P-((D-A))
      | P-((D-A)*B)
      | P-((D-A)*B+CARRYIN)
      | P-((D-A)*BCIN)
      | P-((D-A)*BCIN+CARRYIN)
      | P-((D-A)+CARRYIN)
      | P-((D-ACIN))
      | P-((D-ACIN)*B)
      | P-((D-ACIN)*B+CARRYIN)
      | P-((D-ACIN)*BCIN)
      | P-((D-ACIN)*BCIN+CARRYIN)
      | P-((D-ACIN)+CARRYIN)
      | P-(A)
      | P-(A*B)
      | P-(A*B+CARRYIN)
      | P-(A*BCIN)
      | P-(A*BCIN+CARRYIN)
      | P-(A+CARRYIN)
      | P-(A+D)
      | P-(A+D)*B
      | P-(A+D)*B-CARRYIN
      | P-(A+D)*BCIN
      | P-(A+D)*BCIN-CARRYIN
      | P-(A+D)-CARRYIN
      | P-(ACIN)
      | P-(ACIN*B)
      | P-(ACIN*B+CARRYIN)
      | P-(ACIN*BCIN)
      | P-(ACIN*BCIN+CARRYIN)
      | P-(ACIN+CARRYIN)
      | P-(ACIN+D)
      | P-(ACIN+D)*B
      | P-(ACIN+D)*B-CARRYIN
      | P-(ACIN+D)*BCIN
      | P-(ACIN+D)*BCIN-CARRYIN
      | P-(ACIN+D)-CARRYIN
      | P-(B*(A+D))
      | P-(B*(A+D)+CARRYIN)
      | P-(B*(ACIN+D))
      | P-(B*(ACIN+D)+CARRYIN)
      | P-(B*(D+A))
      | P-(B*(D+A)+CARRYIN)
      | P-(B*(D+ACIN))
      | P-(B*(D+ACIN)+CARRYIN)
      | P-(B*(D-A))
      | P-(B*(D-A)+CARRYIN)
      | P-(B*(D-ACIN))
      | P-(B*(D-ACIN)+CARRYIN)
      | P-(B*A)
      | P-(B*A+CARRYIN)
      | P-(B*ACIN)
      | P-(B*ACIN+CARRYIN)
      | P-(B*D)
      | P-(B*D+CARRYIN)
      | P-(BCIN*(A+D))
      | P-(BCIN*(A+D)+CARRYIN)
      | P-(BCIN*(ACIN+D))
      | P-(BCIN*(ACIN+D)+CARRYIN)
      | P-(BCIN*(D+A))
      | P-(BCIN*(D+A)+CARRYIN)
      | P-(BCIN*(D+ACIN))
      | P-(BCIN*(D+ACIN)+CARRYIN)
      | P-(BCIN*(D-A))
      | P-(BCIN*(D-A)+CARRYIN)
      | P-(BCIN*(D-ACIN))
      | P-(BCIN*(D-ACIN)+CARRYIN)
      | P-(BCIN*A)
      | P-(BCIN*A+CARRYIN)
      | P-(BCIN*ACIN)
      | P-(BCIN*ACIN+CARRYIN)
      | P-(BCIN*D)
      | P-(BCIN*D+CARRYIN)
      | P-(C)
      | P-(C+CARRYCASCIN)
      | P-(C+CARRYIN)
      | P-(C+CONCAT)
      | P-(C+CONCAT+CARRYIN)
      | P-(C+P)
      | P-(C+P+CARRYIN)
      | P-(CARRYCASCIN)
      | P-(CARRYIN)
      | P-(CONCAT)
      | P-(CONCAT+C)
      | P-(CONCAT+C+CARRYIN)
      | P-(CONCAT+CARRYCASCIN)
      | P-(CONCAT+CARRYIN)
      | P-(D)
      | P-(D*B)
      | P-(D*B+CARRYIN)
      | P-(D*BCIN)
      | P-(D*BCIN+CARRYIN)
      | P-(D+A)
      | P-(D+A)*B
      | P-(D+A)*B-CARRYIN
      | P-(D+A)*BCIN
      | P-(D+A)*BCIN-CARRYIN
      | P-(D+A)-CARRYIN
      | P-(D+ACIN)
      | P-(D+ACIN)*B
      | P-(D+ACIN)*B-CARRYIN
      | P-(D+ACIN)*BCIN
      | P-(D+ACIN)*BCIN-CARRYIN
      | P-(D+ACIN)-CARRYIN
      | P-(D+CARRYIN)
      | P-(D-A)
      | P-(D-A)*B
      | P-(D-A)*B-CARRYIN
      | P-(D-A)*BCIN
      | P-(D-A)*BCIN-CARRYIN
      | P-(D-A)-CARRYIN
      | P-(D-ACIN)
      | P-(D-ACIN)*B
      | P-(D-ACIN)*B-CARRYIN
      | P-(D-ACIN)*BCIN
      | P-(D-ACIN)*BCIN-CARRYIN
      | P-(D-ACIN)-CARRYIN
      | P-(P)
      | P-(P+C)
      | P-(P+C+CARRYIN)
      | P-(P+CARRYCASCIN)
      | P-(P+CARRYIN)
      | P-A
      | P-A*B
      | P-A*B-CARRYIN
      | P-A*BCIN
      | P-A*BCIN-CARRYIN
      | P-A-CARRYIN
      | P-ACIN
      | P-ACIN*B
      | P-ACIN*B-CARRYIN
      | P-ACIN*BCIN
      | P-ACIN*BCIN-CARRYIN
      | P-ACIN-CARRYIN
      | P-B*(A+D)
      | P-B*(A+D)-CARRYIN
      | P-B*(ACIN+D)
      | P-B*(ACIN+D)-CARRYIN
      | P-B*(D+A)
      | P-B*(D+A)-CARRYIN
      | P-B*(D+ACIN)
      | P-B*(D+ACIN)-CARRYIN
      | P-B*(D-A)
      | P-B*(D-A)-CARRYIN
      | P-B*(D-ACIN)
      | P-B*(D-ACIN)-CARRYIN
      | P-B*A
      | P-B*A-CARRYIN
      | P-B*ACIN
      | P-B*ACIN-CARRYIN
      | P-B*D
      | P-B*D-CARRYIN
      | P-BCIN*(A+D)
      | P-BCIN*(A+D)-CARRYIN
      | P-BCIN*(ACIN+D)
      | P-BCIN*(ACIN+D)-CARRYIN
      | P-BCIN*(D+A)
      | P-BCIN*(D+A)-CARRYIN
      | P-BCIN*(D+ACIN)
      | P-BCIN*(D+ACIN)-CARRYIN
      | P-BCIN*(D-A)
      | P-BCIN*(D-A)-CARRYIN
      | P-BCIN*(D-ACIN)
      | P-BCIN*(D-ACIN)-CARRYIN
      | P-BCIN*A
      | P-BCIN*A-CARRYIN
      | P-BCIN*ACIN
      | P-BCIN*ACIN-CARRYIN
      | P-BCIN*D
      | P-BCIN*D-CARRYIN
      | P-C
      | P-C-CARRYCASCIN
      | P-C-CARRYIN
      | P-C-CONCAT
      | P-C-CONCAT-CARRYIN
      | P-C-P
      | P-C-P-CARRYIN
      | P-CARRYCASCIN
      | P-CARRYIN
      | P-CONCAT
      | P-CONCAT-C
      | P-CONCAT-C-CARRYIN
      | P-CONCAT-CARRYCASCIN
      | P-CONCAT-CARRYIN
      | P-D
      | P-D*B
      | P-D*B-CARRYIN
      | P-D*BCIN
      | P-D*BCIN-CARRYIN
      | P-D-CARRYIN
      | P-P
      | P-P-C
      | P-P-C-CARRYIN
      | P-P-CARRYCASCIN
      | P-P-CARRYIN
      | P>>17
      | P>>17+(A+D)
      | P>>17+(A+D)*B
      | P>>17+(A+D)*B+CARRYIN
      | P>>17+(A+D)*BCIN
      | P>>17+(A+D)*BCIN+CARRYIN
      | P>>17+(A+D)+CARRYIN
      | P>>17+(ACIN+D)
      | P>>17+(ACIN+D)*B
      | P>>17+(ACIN+D)*B+CARRYIN
      | P>>17+(ACIN+D)*BCIN
      | P>>17+(ACIN+D)*BCIN+CARRYIN
      | P>>17+(ACIN+D)+CARRYIN
      | P>>17+(D+A)
      | P>>17+(D+A)*B
      | P>>17+(D+A)*B+CARRYIN
      | P>>17+(D+A)*BCIN
      | P>>17+(D+A)*BCIN+CARRYIN
      | P>>17+(D+A)+CARRYIN
      | P>>17+(D+ACIN)
      | P>>17+(D+ACIN)*B
      | P>>17+(D+ACIN)*B+CARRYIN
      | P>>17+(D+ACIN)*BCIN
      | P>>17+(D+ACIN)*BCIN+CARRYIN
      | P>>17+(D+ACIN)+CARRYIN
      | P>>17+(D-A)
      | P>>17+(D-A)*B
      | P>>17+(D-A)*B+CARRYIN
      | P>>17+(D-A)*BCIN
      | P>>17+(D-A)*BCIN+CARRYIN
      | P>>17+(D-A)+CARRYIN
      | P>>17+(D-ACIN)
      | P>>17+(D-ACIN)*B
      | P>>17+(D-ACIN)*B+CARRYIN
      | P>>17+(D-ACIN)*BCIN
      | P>>17+(D-ACIN)*BCIN+CARRYIN
      | P>>17+(D-ACIN)+CARRYIN
      | P>>17+A
      | P>>17+A*B
      | P>>17+A*B+CARRYIN
      | P>>17+A*BCIN
      | P>>17+A*BCIN+CARRYIN
      | P>>17+A+CARRYIN
      | P>>17+ACIN
      | P>>17+ACIN*B
      | P>>17+ACIN*B+CARRYIN
      | P>>17+ACIN*BCIN
      | P>>17+ACIN*BCIN+CARRYIN
      | P>>17+ACIN+CARRYIN
      | P>>17+B*(A+D)
      | P>>17+B*(A+D)+CARRYIN
      | P>>17+B*(ACIN+D)
      | P>>17+B*(ACIN+D)+CARRYIN
      | P>>17+B*(D+A)
      | P>>17+B*(D+A)+CARRYIN
      | P>>17+B*(D+ACIN)
      | P>>17+B*(D+ACIN)+CARRYIN
      | P>>17+B*(D-A)
      | P>>17+B*(D-A)+CARRYIN
      | P>>17+B*(D-ACIN)
      | P>>17+B*(D-ACIN)+CARRYIN
      | P>>17+B*A
      | P>>17+B*A+CARRYIN
      | P>>17+B*ACIN
      | P>>17+B*ACIN+CARRYIN
      | P>>17+B*D
      | P>>17+B*D+CARRYIN
      | P>>17+BCIN*(A+D)
      | P>>17+BCIN*(A+D)+CARRYIN
      | P>>17+BCIN*(ACIN+D)
      | P>>17+BCIN*(ACIN+D)+CARRYIN
      | P>>17+BCIN*(D+A)
      | P>>17+BCIN*(D+A)+CARRYIN
      | P>>17+BCIN*(D+ACIN)
      | P>>17+BCIN*(D+ACIN)+CARRYIN
      | P>>17+BCIN*(D-A)
      | P>>17+BCIN*(D-A)+CARRYIN
      | P>>17+BCIN*(D-ACIN)
      | P>>17+BCIN*(D-ACIN)+CARRYIN
      | P>>17+BCIN*A
      | P>>17+BCIN*A+CARRYIN
      | P>>17+BCIN*ACIN
      | P>>17+BCIN*ACIN+CARRYIN
      | P>>17+BCIN*D
      | P>>17+BCIN*D+CARRYIN
      | P>>17+C
      | P>>17+C+CARRYIN
      | P>>17+C+CONCAT
      | P>>17+C+CONCAT+CARRYIN
      | P>>17+C+P
      | P>>17+C+P+CARRYIN
      | P>>17+CARRYIN
      | P>>17+CONCAT
      | P>>17+CONCAT+C
      | P>>17+CONCAT+C+CARRYIN
      | P>>17+CONCAT+CARRYIN
      | P>>17+D
      | P>>17+D*B
      | P>>17+D*B+CARRYIN
      | P>>17+D*BCIN
      | P>>17+D*BCIN+CARRYIN
      | P>>17+D+CARRYIN
      | P>>17+P
      | P>>17+P+C
      | P>>17+P+C+CARRYIN
      | P>>17+P+CARRYIN
      | P>>17-((A+D))
      | P>>17-((A+D)*B)
      | P>>17-((A+D)*B+CARRYIN)
      | P>>17-((A+D)*BCIN)
      | P>>17-((A+D)*BCIN+CARRYIN)
      | P>>17-((A+D)+CARRYIN)
      | P>>17-((ACIN+D))
      | P>>17-((ACIN+D)*B)
      | P>>17-((ACIN+D)*B+CARRYIN)
      | P>>17-((ACIN+D)*BCIN)
      | P>>17-((ACIN+D)*BCIN+CARRYIN)
      | P>>17-((ACIN+D)+CARRYIN)
      | P>>17-((D+A))
      | P>>17-((D+A)*B)
      | P>>17-((D+A)*B+CARRYIN)
      | P>>17-((D+A)*BCIN)
      | P>>17-((D+A)*BCIN+CARRYIN)
      | P>>17-((D+A)+CARRYIN)
      | P>>17-((D+ACIN))
      | P>>17-((D+ACIN)*B)
      | P>>17-((D+ACIN)*B+CARRYIN)
      | P>>17-((D+ACIN)*BCIN)
      | P>>17-((D+ACIN)*BCIN+CARRYIN)
      | P>>17-((D+ACIN)+CARRYIN)
      | P>>17-((D-A))
      | P>>17-((D-A)*B)
      | P>>17-((D-A)*B+CARRYIN)
      | P>>17-((D-A)*BCIN)
      | P>>17-((D-A)*BCIN+CARRYIN)
      | P>>17-((D-A)+CARRYIN)
      | P>>17-((D-ACIN))
      | P>>17-((D-ACIN)*B)
      | P>>17-((D-ACIN)*B+CARRYIN)
      | P>>17-((D-ACIN)*BCIN)
      | P>>17-((D-ACIN)*BCIN+CARRYIN)
      | P>>17-((D-ACIN)+CARRYIN)
      | P>>17-(A)
      | P>>17-(A*B)
      | P>>17-(A*B+CARRYIN)
      | P>>17-(A*BCIN)
      | P>>17-(A*BCIN+CARRYIN)
      | P>>17-(A+CARRYIN)
      | P>>17-(A+D)
      | P>>17-(A+D)*B
      | P>>17-(A+D)*B-CARRYIN
      | P>>17-(A+D)*BCIN
      | P>>17-(A+D)*BCIN-CARRYIN
      | P>>17-(A+D)-CARRYIN
      | P>>17-(ACIN)
      | P>>17-(ACIN*B)
      | P>>17-(ACIN*B+CARRYIN)
      | P>>17-(ACIN*BCIN)
      | P>>17-(ACIN*BCIN+CARRYIN)
      | P>>17-(ACIN+CARRYIN)
      | P>>17-(ACIN+D)
      | P>>17-(ACIN+D)*B
      | P>>17-(ACIN+D)*B-CARRYIN
      | P>>17-(ACIN+D)*BCIN
      | P>>17-(ACIN+D)*BCIN-CARRYIN
      | P>>17-(ACIN+D)-CARRYIN
      | P>>17-(B*(A+D))
      | P>>17-(B*(A+D)+CARRYIN)
      | P>>17-(B*(ACIN+D))
      | P>>17-(B*(ACIN+D)+CARRYIN)
      | P>>17-(B*(D+A))
      | P>>17-(B*(D+A)+CARRYIN)
      | P>>17-(B*(D+ACIN))
      | P>>17-(B*(D+ACIN)+CARRYIN)
      | P>>17-(B*(D-A))
      | P>>17-(B*(D-A)+CARRYIN)
      | P>>17-(B*(D-ACIN))
      | P>>17-(B*(D-ACIN)+CARRYIN)
      | P>>17-(B*A)
      | P>>17-(B*A+CARRYIN)
      | P>>17-(B*ACIN)
      | P>>17-(B*ACIN+CARRYIN)
      | P>>17-(B*D)
      | P>>17-(B*D+CARRYIN)
      | P>>17-(BCIN*(A+D))
      | P>>17-(BCIN*(A+D)+CARRYIN)
      | P>>17-(BCIN*(ACIN+D))
      | P>>17-(BCIN*(ACIN+D)+CARRYIN)
      | P>>17-(BCIN*(D+A))
      | P>>17-(BCIN*(D+A)+CARRYIN)
      | P>>17-(BCIN*(D+ACIN))
      | P>>17-(BCIN*(D+ACIN)+CARRYIN)
      | P>>17-(BCIN*(D-A))
      | P>>17-(BCIN*(D-A)+CARRYIN)
      | P>>17-(BCIN*(D-ACIN))
      | P>>17-(BCIN*(D-ACIN)+CARRYIN)
      | P>>17-(BCIN*A)
      | P>>17-(BCIN*A+CARRYIN)
      | P>>17-(BCIN*ACIN)
      | P>>17-(BCIN*ACIN+CARRYIN)
      | P>>17-(BCIN*D)
      | P>>17-(BCIN*D+CARRYIN)
      | P>>17-(C)
      | P>>17-(C+CARRYIN)
      | P>>17-(C+CONCAT)
      | P>>17-(C+CONCAT+CARRYIN)
      | P>>17-(C+P)
      | P>>17-(C+P+CARRYIN)
      | P>>17-(CARRYIN)
      | P>>17-(CONCAT)
      | P>>17-(CONCAT+C)
      | P>>17-(CONCAT+C+CARRYIN)
      | P>>17-(CONCAT+CARRYIN)
      | P>>17-(D)
      | P>>17-(D*B)
      | P>>17-(D*B+CARRYIN)
      | P>>17-(D*BCIN)
      | P>>17-(D*BCIN+CARRYIN)
      | P>>17-(D+A)
      | P>>17-(D+A)*B
      | P>>17-(D+A)*B-CARRYIN
      | P>>17-(D+A)*BCIN
      | P>>17-(D+A)*BCIN-CARRYIN
      | P>>17-(D+A)-CARRYIN
      | P>>17-(D+ACIN)
      | P>>17-(D+ACIN)*B
      | P>>17-(D+ACIN)*B-CARRYIN
      | P>>17-(D+ACIN)*BCIN
      | P>>17-(D+ACIN)*BCIN-CARRYIN
      | P>>17-(D+ACIN)-CARRYIN
      | P>>17-(D+CARRYIN)
      | P>>17-(D-A)
      | P>>17-(D-A)*B
      | P>>17-(D-A)*B-CARRYIN
      | P>>17-(D-A)*BCIN
      | P>>17-(D-A)*BCIN-CARRYIN
      | P>>17-(D-A)-CARRYIN
      | P>>17-(D-ACIN)
      | P>>17-(D-ACIN)*B
      | P>>17-(D-ACIN)*B-CARRYIN
      | P>>17-(D-ACIN)*BCIN
      | P>>17-(D-ACIN)*BCIN-CARRYIN
      | P>>17-(D-ACIN)-CARRYIN
      | P>>17-(P)
      | P>>17-(P+C)
      | P>>17-(P+C+CARRYIN)
      | P>>17-(P+CARRYIN)
      | P>>17-A
      | P>>17-A*B
      | P>>17-A*B-CARRYIN
      | P>>17-A*BCIN
      | P>>17-A*BCIN-CARRYIN
      | P>>17-A-CARRYIN
      | P>>17-ACIN
      | P>>17-ACIN*B
      | P>>17-ACIN*B-CARRYIN
      | P>>17-ACIN*BCIN
      | P>>17-ACIN*BCIN-CARRYIN
      | P>>17-ACIN-CARRYIN
      | P>>17-B*(A+D)
      | P>>17-B*(A+D)-CARRYIN
      | P>>17-B*(ACIN+D)
      | P>>17-B*(ACIN+D)-CARRYIN
      | P>>17-B*(D+A)
      | P>>17-B*(D+A)-CARRYIN
      | P>>17-B*(D+ACIN)
      | P>>17-B*(D+ACIN)-CARRYIN
      | P>>17-B*(D-A)
      | P>>17-B*(D-A)-CARRYIN
      | P>>17-B*(D-ACIN)
      | P>>17-B*(D-ACIN)-CARRYIN
      | P>>17-B*A
      | P>>17-B*A-CARRYIN
      | P>>17-B*ACIN
      | P>>17-B*ACIN-CARRYIN
      | P>>17-B*D
      | P>>17-B*D-CARRYIN
      | P>>17-BCIN*(A+D)
      | P>>17-BCIN*(A+D)-CARRYIN
      | P>>17-BCIN*(ACIN+D)
      | P>>17-BCIN*(ACIN+D)-CARRYIN
      | P>>17-BCIN*(D+A)
      | P>>17-BCIN*(D+A)-CARRYIN
      | P>>17-BCIN*(D+ACIN)
      | P>>17-BCIN*(D+ACIN)-CARRYIN
      | P>>17-BCIN*(D-A)
      | P>>17-BCIN*(D-A)-CARRYIN
      | P>>17-BCIN*(D-ACIN)
      | P>>17-BCIN*(D-ACIN)-CARRYIN
      | P>>17-BCIN*A
      | P>>17-BCIN*A-CARRYIN
      | P>>17-BCIN*ACIN
      | P>>17-BCIN*ACIN-CARRYIN
      | P>>17-BCIN*D
      | P>>17-BCIN*D-CARRYIN
      | P>>17-C
      | P>>17-C-CARRYIN
      | P>>17-C-CONCAT
      | P>>17-C-CONCAT-CARRYIN
      | P>>17-C-P
      | P>>17-C-P-CARRYIN
      | P>>17-CARRYIN
      | P>>17-CONCAT
      | P>>17-CONCAT-C
      | P>>17-CONCAT-C-CARRYIN
      | P>>17-CONCAT-CARRYIN
      | P>>17-D
      | P>>17-D*B
      | P>>17-D*B-CARRYIN
      | P>>17-D*BCIN
      | P>>17-D*BCIN-CARRYIN
      | P>>17-D-CARRYIN
      | P>>17-P
      | P>>17-P-C
      | P>>17-P-C-CARRYIN
      | P>>17-P-CARRYIN
      | PCIN
      | PCIN+(A+D)
      | PCIN+(A+D)*B
      | PCIN+(A+D)*B+CARRYIN
      | PCIN+(A+D)*BCIN
      | PCIN+(A+D)*BCIN+CARRYIN
      | PCIN+(A+D)+CARRYIN
      | PCIN+(ACIN+D)
      | PCIN+(ACIN+D)*B
      | PCIN+(ACIN+D)*B+CARRYIN
      | PCIN+(ACIN+D)*BCIN
      | PCIN+(ACIN+D)*BCIN+CARRYIN
      | PCIN+(ACIN+D)+CARRYIN
      | PCIN+(D+A)
      | PCIN+(D+A)*B
      | PCIN+(D+A)*B+CARRYIN
      | PCIN+(D+A)*BCIN
      | PCIN+(D+A)*BCIN+CARRYIN
      | PCIN+(D+A)+CARRYIN
      | PCIN+(D+ACIN)
      | PCIN+(D+ACIN)*B
      | PCIN+(D+ACIN)*B+CARRYIN
      | PCIN+(D+ACIN)*BCIN
      | PCIN+(D+ACIN)*BCIN+CARRYIN
      | PCIN+(D+ACIN)+CARRYIN
      | PCIN+(D-A)
      | PCIN+(D-A)*B
      | PCIN+(D-A)*B+CARRYIN
      | PCIN+(D-A)*BCIN
      | PCIN+(D-A)*BCIN+CARRYIN
      | PCIN+(D-A)+CARRYIN
      | PCIN+(D-ACIN)
      | PCIN+(D-ACIN)*B
      | PCIN+(D-ACIN)*B+CARRYIN
      | PCIN+(D-ACIN)*BCIN
      | PCIN+(D-ACIN)*BCIN+CARRYIN
      | PCIN+(D-ACIN)+CARRYIN
      | PCIN+A
      | PCIN+A*B
      | PCIN+A*B+CARRYIN
      | PCIN+A*BCIN
      | PCIN+A*BCIN+CARRYIN
      | PCIN+A+CARRYIN
      | PCIN+ACIN
      | PCIN+ACIN*B
      | PCIN+ACIN*B+CARRYIN
      | PCIN+ACIN*BCIN
      | PCIN+ACIN*BCIN+CARRYIN
      | PCIN+ACIN+CARRYIN
      | PCIN+B*(A+D)
      | PCIN+B*(A+D)+CARRYIN
      | PCIN+B*(ACIN+D)
      | PCIN+B*(ACIN+D)+CARRYIN
      | PCIN+B*(D+A)
      | PCIN+B*(D+A)+CARRYIN
      | PCIN+B*(D+ACIN)
      | PCIN+B*(D+ACIN)+CARRYIN
      | PCIN+B*(D-A)
      | PCIN+B*(D-A)+CARRYIN
      | PCIN+B*(D-ACIN)
      | PCIN+B*(D-ACIN)+CARRYIN
      | PCIN+B*A
      | PCIN+B*A+CARRYIN
      | PCIN+B*ACIN
      | PCIN+B*ACIN+CARRYIN
      | PCIN+B*D
      | PCIN+B*D+CARRYIN
      | PCIN+BCIN*(A+D)
      | PCIN+BCIN*(A+D)+CARRYIN
      | PCIN+BCIN*(ACIN+D)
      | PCIN+BCIN*(ACIN+D)+CARRYIN
      | PCIN+BCIN*(D+A)
      | PCIN+BCIN*(D+A)+CARRYIN
      | PCIN+BCIN*(D+ACIN)
      | PCIN+BCIN*(D+ACIN)+CARRYIN
      | PCIN+BCIN*(D-A)
      | PCIN+BCIN*(D-A)+CARRYIN
      | PCIN+BCIN*(D-ACIN)
      | PCIN+BCIN*(D-ACIN)+CARRYIN
      | PCIN+BCIN*A
      | PCIN+BCIN*A+CARRYIN
      | PCIN+BCIN*ACIN
      | PCIN+BCIN*ACIN+CARRYIN
      | PCIN+BCIN*D
      | PCIN+BCIN*D+CARRYIN
      | PCIN+C
      | PCIN+C+CARRYIN
      | PCIN+C+CONCAT
      | PCIN+C+CONCAT+CARRYIN
      | PCIN+C+P
      | PCIN+C+P+CARRYIN
      | PCIN+CARRYIN
      | PCIN+CONCAT
      | PCIN+CONCAT+C
      | PCIN+CONCAT+C+CARRYIN
      | PCIN+CONCAT+CARRYIN
      | PCIN+D
      | PCIN+D*B
      | PCIN+D*B+CARRYIN
      | PCIN+D*BCIN
      | PCIN+D*BCIN+CARRYIN
      | PCIN+D+CARRYIN
      | PCIN+P
      | PCIN+P+C
      | PCIN+P+C+CARRYIN
      | PCIN+P+CARRYIN
      | PCIN-((A+D))
      | PCIN-((A+D)*B)
      | PCIN-((A+D)*B+CARRYIN)
      | PCIN-((A+D)*BCIN)
      | PCIN-((A+D)*BCIN+CARRYIN)
      | PCIN-((A+D)+CARRYIN)
      | PCIN-((ACIN+D))
      | PCIN-((ACIN+D)*B)
      | PCIN-((ACIN+D)*B+CARRYIN)
      | PCIN-((ACIN+D)*BCIN)
      | PCIN-((ACIN+D)*BCIN+CARRYIN)
      | PCIN-((ACIN+D)+CARRYIN)
      | PCIN-((D+A))
      | PCIN-((D+A)*B)
      | PCIN-((D+A)*B+CARRYIN)
      | PCIN-((D+A)*BCIN)
      | PCIN-((D+A)*BCIN+CARRYIN)
      | PCIN-((D+A)+CARRYIN)
      | PCIN-((D+ACIN))
      | PCIN-((D+ACIN)*B)
      | PCIN-((D+ACIN)*B+CARRYIN)
      | PCIN-((D+ACIN)*BCIN)
      | PCIN-((D+ACIN)*BCIN+CARRYIN)
      | PCIN-((D+ACIN)+CARRYIN)
      | PCIN-((D-A))
      | PCIN-((D-A)*B)
      | PCIN-((D-A)*B+CARRYIN)
      | PCIN-((D-A)*BCIN)
      | PCIN-((D-A)*BCIN+CARRYIN)
      | PCIN-((D-A)+CARRYIN)
      | PCIN-((D-ACIN))
      | PCIN-((D-ACIN)*B)
      | PCIN-((D-ACIN)*B+CARRYIN)
      | PCIN-((D-ACIN)*BCIN)
      | PCIN-((D-ACIN)*BCIN+CARRYIN)
      | PCIN-((D-ACIN)+CARRYIN)
      | PCIN-(A)
      | PCIN-(A*B)
      | PCIN-(A*B+CARRYIN)
      | PCIN-(A*BCIN)
      | PCIN-(A*BCIN+CARRYIN)
      | PCIN-(A+CARRYIN)
      | PCIN-(A+D)
      | PCIN-(A+D)*B
      | PCIN-(A+D)*B-CARRYIN
      | PCIN-(A+D)*BCIN
      | PCIN-(A+D)*BCIN-CARRYIN
      | PCIN-(A+D)-CARRYIN
      | PCIN-(ACIN)
      | PCIN-(ACIN*B)
      | PCIN-(ACIN*B+CARRYIN)
      | PCIN-(ACIN*BCIN)
      | PCIN-(ACIN*BCIN+CARRYIN)
      | PCIN-(ACIN+CARRYIN)
      | PCIN-(ACIN+D)
      | PCIN-(ACIN+D)*B
      | PCIN-(ACIN+D)*B-CARRYIN
      | PCIN-(ACIN+D)*BCIN
      | PCIN-(ACIN+D)*BCIN-CARRYIN
      | PCIN-(ACIN+D)-CARRYIN
      | PCIN-(B*(A+D))
      | PCIN-(B*(A+D)+CARRYIN)
      | PCIN-(B*(ACIN+D))
      | PCIN-(B*(ACIN+D)+CARRYIN)
      | PCIN-(B*(D+A))
      | PCIN-(B*(D+A)+CARRYIN)
      | PCIN-(B*(D+ACIN))
      | PCIN-(B*(D+ACIN)+CARRYIN)
      | PCIN-(B*(D-A))
      | PCIN-(B*(D-A)+CARRYIN)
      | PCIN-(B*(D-ACIN))
      | PCIN-(B*(D-ACIN)+CARRYIN)
      | PCIN-(B*A)
      | PCIN-(B*A+CARRYIN)
      | PCIN-(B*ACIN)
      | PCIN-(B*ACIN+CARRYIN)
      | PCIN-(B*D)
      | PCIN-(B*D+CARRYIN)
      | PCIN-(BCIN*(A+D))
      | PCIN-(BCIN*(A+D)+CARRYIN)
      | PCIN-(BCIN*(ACIN+D))
      | PCIN-(BCIN*(ACIN+D)+CARRYIN)
      | PCIN-(BCIN*(D+A))
      | PCIN-(BCIN*(D+A)+CARRYIN)
      | PCIN-(BCIN*(D+ACIN))
      | PCIN-(BCIN*(D+ACIN)+CARRYIN)
      | PCIN-(BCIN*(D-A))
      | PCIN-(BCIN*(D-A)+CARRYIN)
      | PCIN-(BCIN*(D-ACIN))
      | PCIN-(BCIN*(D-ACIN)+CARRYIN)
      | PCIN-(BCIN*A)
      | PCIN-(BCIN*A+CARRYIN)
      | PCIN-(BCIN*ACIN)
      | PCIN-(BCIN*ACIN+CARRYIN)
      | PCIN-(BCIN*D)
      | PCIN-(BCIN*D+CARRYIN)
      | PCIN-(C)
      | PCIN-(C+CARRYIN)
      | PCIN-(C+CONCAT)
      | PCIN-(C+CONCAT+CARRYIN)
      | PCIN-(C+P)
      | PCIN-(C+P+CARRYIN)
      | PCIN-(CARRYIN)
      | PCIN-(CONCAT)
      | PCIN-(CONCAT+C)
      | PCIN-(CONCAT+C+CARRYIN)
      | PCIN-(CONCAT+CARRYIN)
      | PCIN-(D)
      | PCIN-(D*B)
      | PCIN-(D*B+CARRYIN)
      | PCIN-(D*BCIN)
      | PCIN-(D*BCIN+CARRYIN)
      | PCIN-(D+A)
      | PCIN-(D+A)*B
      | PCIN-(D+A)*B-CARRYIN
      | PCIN-(D+A)*BCIN
      | PCIN-(D+A)*BCIN-CARRYIN
      | PCIN-(D+A)-CARRYIN
      | PCIN-(D+ACIN)
      | PCIN-(D+ACIN)*B
      | PCIN-(D+ACIN)*B-CARRYIN
      | PCIN-(D+ACIN)*BCIN
      | PCIN-(D+ACIN)*BCIN-CARRYIN
      | PCIN-(D+ACIN)-CARRYIN
      | PCIN-(D+CARRYIN)
      | PCIN-(D-A)
      | PCIN-(D-A)*B
      | PCIN-(D-A)*B-CARRYIN
      | PCIN-(D-A)*BCIN
      | PCIN-(D-A)*BCIN-CARRYIN
      | PCIN-(D-A)-CARRYIN
      | PCIN-(D-ACIN)
      | PCIN-(D-ACIN)*B
      | PCIN-(D-ACIN)*B-CARRYIN
      | PCIN-(D-ACIN)*BCIN
      | PCIN-(D-ACIN)*BCIN-CARRYIN
      | PCIN-(D-ACIN)-CARRYIN
      | PCIN-(P)
      | PCIN-(P+C)
      | PCIN-(P+C+CARRYIN)
      | PCIN-(P+CARRYIN)
      | PCIN-A
      | PCIN-A*B
      | PCIN-A*B-CARRYIN
      | PCIN-A*BCIN
      | PCIN-A*BCIN-CARRYIN
      | PCIN-A-CARRYIN
      | PCIN-ACIN
      | PCIN-ACIN*B
      | PCIN-ACIN*B-CARRYIN
      | PCIN-ACIN*BCIN
      | PCIN-ACIN*BCIN-CARRYIN
      | PCIN-ACIN-CARRYIN
      | PCIN-B*(A+D)
      | PCIN-B*(A+D)-CARRYIN
      | PCIN-B*(ACIN+D)
      | PCIN-B*(ACIN+D)-CARRYIN
      | PCIN-B*(D+A)
      | PCIN-B*(D+A)-CARRYIN
      | PCIN-B*(D+ACIN)
      | PCIN-B*(D+ACIN)-CARRYIN
      | PCIN-B*(D-A)
      | PCIN-B*(D-A)-CARRYIN
      | PCIN-B*(D-ACIN)
      | PCIN-B*(D-ACIN)-CARRYIN
      | PCIN-B*A
      | PCIN-B*A-CARRYIN
      | PCIN-B*ACIN
      | PCIN-B*ACIN-CARRYIN
      | PCIN-B*D
      | PCIN-B*D-CARRYIN
      | PCIN-BCIN*(A+D)
      | PCIN-BCIN*(A+D)-CARRYIN
      | PCIN-BCIN*(ACIN+D)
      | PCIN-BCIN*(ACIN+D)-CARRYIN
      | PCIN-BCIN*(D+A)
      | PCIN-BCIN*(D+A)-CARRYIN
      | PCIN-BCIN*(D+ACIN)
      | PCIN-BCIN*(D+ACIN)-CARRYIN
      | PCIN-BCIN*(D-A)
      | PCIN-BCIN*(D-A)-CARRYIN
      | PCIN-BCIN*(D-ACIN)
      | PCIN-BCIN*(D-ACIN)-CARRYIN
      | PCIN-BCIN*A
      | PCIN-BCIN*A-CARRYIN
      | PCIN-BCIN*ACIN
      | PCIN-BCIN*ACIN-CARRYIN
      | PCIN-BCIN*D
      | PCIN-BCIN*D-CARRYIN
      | PCIN-C
      | PCIN-C-CARRYIN
      | PCIN-C-CONCAT
      | PCIN-C-CONCAT-CARRYIN
      | PCIN-C-P
      | PCIN-C-P-CARRYIN
      | PCIN-CARRYIN
      | PCIN-CONCAT
      | PCIN-CONCAT-C
      | PCIN-CONCAT-C-CARRYIN
      | PCIN-CONCAT-CARRYIN
      | PCIN-D
      | PCIN-D*B
      | PCIN-D*B-CARRYIN
      | PCIN-D*BCIN
      | PCIN-D*BCIN-CARRYIN
      | PCIN-D-CARRYIN
      | PCIN-P
      | PCIN-P-C
      | PCIN-P-C-CARRYIN
      | PCIN-P-CARRYIN
      | PCIN>>17
      | PCIN>>17+(A+D)
      | PCIN>>17+(A+D)*B
      | PCIN>>17+(A+D)*B+CARRYIN
      | PCIN>>17+(A+D)*BCIN
      | PCIN>>17+(A+D)*BCIN+CARRYIN
      | PCIN>>17+(A+D)+CARRYIN
      | PCIN>>17+(ACIN+D)
      | PCIN>>17+(ACIN+D)*B
      | PCIN>>17+(ACIN+D)*B+CARRYIN
      | PCIN>>17+(ACIN+D)*BCIN
      | PCIN>>17+(ACIN+D)*BCIN+CARRYIN
      | PCIN>>17+(ACIN+D)+CARRYIN
      | PCIN>>17+(D+A)
      | PCIN>>17+(D+A)*B
      | PCIN>>17+(D+A)*B+CARRYIN
      | PCIN>>17+(D+A)*BCIN
      | PCIN>>17+(D+A)*BCIN+CARRYIN
      | PCIN>>17+(D+A)+CARRYIN
      | PCIN>>17+(D+ACIN)
      | PCIN>>17+(D+ACIN)*B
      | PCIN>>17+(D+ACIN)*B+CARRYIN
      | PCIN>>17+(D+ACIN)*BCIN
      | PCIN>>17+(D+ACIN)*BCIN+CARRYIN
      | PCIN>>17+(D+ACIN)+CARRYIN
      | PCIN>>17+(D-A)
      | PCIN>>17+(D-A)*B
      | PCIN>>17+(D-A)*B+CARRYIN
      | PCIN>>17+(D-A)*BCIN
      | PCIN>>17+(D-A)*BCIN+CARRYIN
      | PCIN>>17+(D-A)+CARRYIN
      | PCIN>>17+(D-ACIN)
      | PCIN>>17+(D-ACIN)*B
      | PCIN>>17+(D-ACIN)*B+CARRYIN
      | PCIN>>17+(D-ACIN)*BCIN
      | PCIN>>17+(D-ACIN)*BCIN+CARRYIN
      | PCIN>>17+(D-ACIN)+CARRYIN
      | PCIN>>17+A
      | PCIN>>17+A*B
      | PCIN>>17+A*B+CARRYIN
      | PCIN>>17+A*BCIN
      | PCIN>>17+A*BCIN+CARRYIN
      | PCIN>>17+A+CARRYIN
      | PCIN>>17+ACIN
      | PCIN>>17+ACIN*B
      | PCIN>>17+ACIN*B+CARRYIN
      | PCIN>>17+ACIN*BCIN
      | PCIN>>17+ACIN*BCIN+CARRYIN
      | PCIN>>17+ACIN+CARRYIN
      | PCIN>>17+B*(A+D)
      | PCIN>>17+B*(A+D)+CARRYIN
      | PCIN>>17+B*(ACIN+D)
      | PCIN>>17+B*(ACIN+D)+CARRYIN
      | PCIN>>17+B*(D+A)
      | PCIN>>17+B*(D+A)+CARRYIN
      | PCIN>>17+B*(D+ACIN)
      | PCIN>>17+B*(D+ACIN)+CARRYIN
      | PCIN>>17+B*(D-A)
      | PCIN>>17+B*(D-A)+CARRYIN
      | PCIN>>17+B*(D-ACIN)
      | PCIN>>17+B*(D-ACIN)+CARRYIN
      | PCIN>>17+B*A
      | PCIN>>17+B*A+CARRYIN
      | PCIN>>17+B*ACIN
      | PCIN>>17+B*ACIN+CARRYIN
      | PCIN>>17+B*D
      | PCIN>>17+B*D+CARRYIN
      | PCIN>>17+BCIN*(A+D)
      | PCIN>>17+BCIN*(A+D)+CARRYIN
      | PCIN>>17+BCIN*(ACIN+D)
      | PCIN>>17+BCIN*(ACIN+D)+CARRYIN
      | PCIN>>17+BCIN*(D+A)
      | PCIN>>17+BCIN*(D+A)+CARRYIN
      | PCIN>>17+BCIN*(D+ACIN)
      | PCIN>>17+BCIN*(D+ACIN)+CARRYIN
      | PCIN>>17+BCIN*(D-A)
      | PCIN>>17+BCIN*(D-A)+CARRYIN
      | PCIN>>17+BCIN*(D-ACIN)
      | PCIN>>17+BCIN*(D-ACIN)+CARRYIN
      | PCIN>>17+BCIN*A
      | PCIN>>17+BCIN*A+CARRYIN
      | PCIN>>17+BCIN*ACIN
      | PCIN>>17+BCIN*ACIN+CARRYIN
      | PCIN>>17+BCIN*D
      | PCIN>>17+BCIN*D+CARRYIN
      | PCIN>>17+C
      | PCIN>>17+C+CARRYIN
      | PCIN>>17+C+CONCAT
      | PCIN>>17+C+CONCAT+CARRYIN
      | PCIN>>17+C+P
      | PCIN>>17+C+P+CARRYIN
      | PCIN>>17+CARRYIN
      | PCIN>>17+CONCAT
      | PCIN>>17+CONCAT+C
      | PCIN>>17+CONCAT+C+CARRYIN
      | PCIN>>17+CONCAT+CARRYIN
      | PCIN>>17+D
      | PCIN>>17+D*B
      | PCIN>>17+D*B+CARRYIN
      | PCIN>>17+D*BCIN
      | PCIN>>17+D*BCIN+CARRYIN
      | PCIN>>17+D+CARRYIN
      | PCIN>>17+P
      | PCIN>>17+P+C
      | PCIN>>17+P+C+CARRYIN
      | PCIN>>17+P+CARRYIN
      | PCIN>>17-((A+D))
      | PCIN>>17-((A+D)*B)
      | PCIN>>17-((A+D)*B+CARRYIN)
      | PCIN>>17-((A+D)*BCIN)
      | PCIN>>17-((A+D)*BCIN+CARRYIN)
      | PCIN>>17-((A+D)+CARRYIN)
      | PCIN>>17-((ACIN+D))
      | PCIN>>17-((ACIN+D)*B)
      | PCIN>>17-((ACIN+D)*B+CARRYIN)
      | PCIN>>17-((ACIN+D)*BCIN)
      | PCIN>>17-((ACIN+D)*BCIN+CARRYIN)
      | PCIN>>17-((ACIN+D)+CARRYIN)
      | PCIN>>17-((D+A))
      | PCIN>>17-((D+A)*B)
      | PCIN>>17-((D+A)*B+CARRYIN)
      | PCIN>>17-((D+A)*BCIN)
      | PCIN>>17-((D+A)*BCIN+CARRYIN)
      | PCIN>>17-((D+A)+CARRYIN)
      | PCIN>>17-((D+ACIN))
      | PCIN>>17-((D+ACIN)*B)
      | PCIN>>17-((D+ACIN)*B+CARRYIN)
      | PCIN>>17-((D+ACIN)*BCIN)
      | PCIN>>17-((D+ACIN)*BCIN+CARRYIN)
      | PCIN>>17-((D+ACIN)+CARRYIN)
      | PCIN>>17-((D-A))
      | PCIN>>17-((D-A)*B)
      | PCIN>>17-((D-A)*B+CARRYIN)
      | PCIN>>17-((D-A)*BCIN)
      | PCIN>>17-((D-A)*BCIN+CARRYIN)
      | PCIN>>17-((D-A)+CARRYIN)
      | PCIN>>17-((D-ACIN))
      | PCIN>>17-((D-ACIN)*B)
      | PCIN>>17-((D-ACIN)*B+CARRYIN)
      | PCIN>>17-((D-ACIN)*BCIN)
      | PCIN>>17-((D-ACIN)*BCIN+CARRYIN)
      | PCIN>>17-((D-ACIN)+CARRYIN)
      | PCIN>>17-(A)
      | PCIN>>17-(A*B)
      | PCIN>>17-(A*B+CARRYIN)
      | PCIN>>17-(A*BCIN)
      | PCIN>>17-(A*BCIN+CARRYIN)
      | PCIN>>17-(A+CARRYIN)
      | PCIN>>17-(A+D)
      | PCIN>>17-(A+D)*B
      | PCIN>>17-(A+D)*B-CARRYIN
      | PCIN>>17-(A+D)*BCIN
      | PCIN>>17-(A+D)*BCIN-CARRYIN
      | PCIN>>17-(A+D)-CARRYIN
      | PCIN>>17-(ACIN)
      | PCIN>>17-(ACIN*B)
      | PCIN>>17-(ACIN*B+CARRYIN)
      | PCIN>>17-(ACIN*BCIN)
      | PCIN>>17-(ACIN*BCIN+CARRYIN)
      | PCIN>>17-(ACIN+CARRYIN)
      | PCIN>>17-(ACIN+D)
      | PCIN>>17-(ACIN+D)*B
      | PCIN>>17-(ACIN+D)*B-CARRYIN
      | PCIN>>17-(ACIN+D)*BCIN
      | PCIN>>17-(ACIN+D)*BCIN-CARRYIN
      | PCIN>>17-(ACIN+D)-CARRYIN
      | PCIN>>17-(B*(A+D))
      | PCIN>>17-(B*(A+D)+CARRYIN)
      | PCIN>>17-(B*(ACIN+D))
      | PCIN>>17-(B*(ACIN+D)+CARRYIN)
      | PCIN>>17-(B*(D+A))
      | PCIN>>17-(B*(D+A)+CARRYIN)
      | PCIN>>17-(B*(D+ACIN))
      | PCIN>>17-(B*(D+ACIN)+CARRYIN)
      | PCIN>>17-(B*(D-A))
      | PCIN>>17-(B*(D-A)+CARRYIN)
      | PCIN>>17-(B*(D-ACIN))
      | PCIN>>17-(B*(D-ACIN)+CARRYIN)
      | PCIN>>17-(B*A)
      | PCIN>>17-(B*A+CARRYIN)
      | PCIN>>17-(B*ACIN)
      | PCIN>>17-(B*ACIN+CARRYIN)
      | PCIN>>17-(B*D)
      | PCIN>>17-(B*D+CARRYIN)
      | PCIN>>17-(BCIN*(A+D))
      | PCIN>>17-(BCIN*(A+D)+CARRYIN)
      | PCIN>>17-(BCIN*(ACIN+D))
      | PCIN>>17-(BCIN*(ACIN+D)+CARRYIN)
      | PCIN>>17-(BCIN*(D+A))
      | PCIN>>17-(BCIN*(D+A)+CARRYIN)
      | PCIN>>17-(BCIN*(D+ACIN))
      | PCIN>>17-(BCIN*(D+ACIN)+CARRYIN)
      | PCIN>>17-(BCIN*(D-A))
      | PCIN>>17-(BCIN*(D-A)+CARRYIN)
      | PCIN>>17-(BCIN*(D-ACIN))
      | PCIN>>17-(BCIN*(D-ACIN)+CARRYIN)
      | PCIN>>17-(BCIN*A)
      | PCIN>>17-(BCIN*A+CARRYIN)
      | PCIN>>17-(BCIN*ACIN)
      | PCIN>>17-(BCIN*ACIN+CARRYIN)
      | PCIN>>17-(BCIN*D)
      | PCIN>>17-(BCIN*D+CARRYIN)
      | PCIN>>17-(C)
      | PCIN>>17-(C+CARRYIN)
      | PCIN>>17-(C+CONCAT)
      | PCIN>>17-(C+CONCAT+CARRYIN)
      | PCIN>>17-(C+P)
      | PCIN>>17-(C+P+CARRYIN)
      | PCIN>>17-(CARRYIN)
      | PCIN>>17-(CONCAT)
      | PCIN>>17-(CONCAT+C)
      | PCIN>>17-(CONCAT+C+CARRYIN)
      | PCIN>>17-(CONCAT+CARRYIN)
      | PCIN>>17-(D)
      | PCIN>>17-(D*B)
      | PCIN>>17-(D*B+CARRYIN)
      | PCIN>>17-(D*BCIN)
      | PCIN>>17-(D*BCIN+CARRYIN)
      | PCIN>>17-(D+A)
      | PCIN>>17-(D+A)*B
      | PCIN>>17-(D+A)*B-CARRYIN
      | PCIN>>17-(D+A)*BCIN
      | PCIN>>17-(D+A)*BCIN-CARRYIN
      | PCIN>>17-(D+A)-CARRYIN
      | PCIN>>17-(D+ACIN)
      | PCIN>>17-(D+ACIN)*B
      | PCIN>>17-(D+ACIN)*B-CARRYIN
      | PCIN>>17-(D+ACIN)*BCIN
      | PCIN>>17-(D+ACIN)*BCIN-CARRYIN
      | PCIN>>17-(D+ACIN)-CARRYIN
      | PCIN>>17-(D+CARRYIN)
      | PCIN>>17-(D-A)
      | PCIN>>17-(D-A)*B
      | PCIN>>17-(D-A)*B-CARRYIN
      | PCIN>>17-(D-A)*BCIN
      | PCIN>>17-(D-A)*BCIN-CARRYIN
      | PCIN>>17-(D-A)-CARRYIN
      | PCIN>>17-(D-ACIN)
      | PCIN>>17-(D-ACIN)*B
      | PCIN>>17-(D-ACIN)*B-CARRYIN
      | PCIN>>17-(D-ACIN)*BCIN
      | PCIN>>17-(D-ACIN)*BCIN-CARRYIN
      | PCIN>>17-(D-ACIN)-CARRYIN
      | PCIN>>17-(P)
      | PCIN>>17-(P+C)
      | PCIN>>17-(P+C+CARRYIN)
      | PCIN>>17-(P+CARRYIN)
      | PCIN>>17-A
      | PCIN>>17-A*B
      | PCIN>>17-A*B-CARRYIN
      | PCIN>>17-A*BCIN
      | PCIN>>17-A*BCIN-CARRYIN
      | PCIN>>17-A-CARRYIN
      | PCIN>>17-ACIN
      | PCIN>>17-ACIN*B
      | PCIN>>17-ACIN*B-CARRYIN
      | PCIN>>17-ACIN*BCIN
      | PCIN>>17-ACIN*BCIN-CARRYIN
      | PCIN>>17-ACIN-CARRYIN
      | PCIN>>17-B*(A+D)
      | PCIN>>17-B*(A+D)-CARRYIN
      | PCIN>>17-B*(ACIN+D)
      | PCIN>>17-B*(ACIN+D)-CARRYIN
      | PCIN>>17-B*(D+A)
      | PCIN>>17-B*(D+A)-CARRYIN
      | PCIN>>17-B*(D+ACIN)
      | PCIN>>17-B*(D+ACIN)-CARRYIN
      | PCIN>>17-B*(D-A)
      | PCIN>>17-B*(D-A)-CARRYIN
      | PCIN>>17-B*(D-ACIN)
      | PCIN>>17-B*(D-ACIN)-CARRYIN
      | PCIN>>17-B*A
      | PCIN>>17-B*A-CARRYIN
      | PCIN>>17-B*ACIN
      | PCIN>>17-B*ACIN-CARRYIN
      | PCIN>>17-B*D
      | PCIN>>17-B*D-CARRYIN
      | PCIN>>17-BCIN*(A+D)
      | PCIN>>17-BCIN*(A+D)-CARRYIN
      | PCIN>>17-BCIN*(ACIN+D)
      | PCIN>>17-BCIN*(ACIN+D)-CARRYIN
      | PCIN>>17-BCIN*(D+A)
      | PCIN>>17-BCIN*(D+A)-CARRYIN
      | PCIN>>17-BCIN*(D+ACIN)
      | PCIN>>17-BCIN*(D+ACIN)-CARRYIN
      | PCIN>>17-BCIN*(D-A)
      | PCIN>>17-BCIN*(D-A)-CARRYIN
      | PCIN>>17-BCIN*(D-ACIN)
      | PCIN>>17-BCIN*(D-ACIN)-CARRYIN
      | PCIN>>17-BCIN*A
      | PCIN>>17-BCIN*A-CARRYIN
      | PCIN>>17-BCIN*ACIN
      | PCIN>>17-BCIN*ACIN-CARRYIN
      | PCIN>>17-BCIN*D
      | PCIN>>17-BCIN*D-CARRYIN
      | PCIN>>17-C
      | PCIN>>17-C-CARRYIN
      | PCIN>>17-C-CONCAT
      | PCIN>>17-C-CONCAT-CARRYIN
      | PCIN>>17-C-P
      | PCIN>>17-C-P-CARRYIN
      | PCIN>>17-CARRYIN
      | PCIN>>17-CONCAT
      | PCIN>>17-CONCAT-C
      | PCIN>>17-CONCAT-C-CARRYIN
      | PCIN>>17-CONCAT-CARRYIN
      | PCIN>>17-D
      | PCIN>>17-D*B
      | PCIN>>17-D*B-CARRYIN
      | PCIN>>17-D*BCIN
      | PCIN>>17-D*BCIN-CARRYIN
      | PCIN>>17-D-CARRYIN
      | PCIN>>17-P
      | PCIN>>17-P-C
      | PCIN>>17-P-C-CARRYIN
      | PCIN>>17-P-CARRYIN
      | RNDSIMPLE((A+D))
      | RNDSIMPLE((A+D)*B)
      | RNDSIMPLE((A+D)*B+CARRYIN)
      | RNDSIMPLE((A+D)*BCIN)
      | RNDSIMPLE((A+D)*BCIN+CARRYIN)
      | RNDSIMPLE((A+D)+CARRYIN)
      | RNDSIMPLE((ACIN+D))
      | RNDSIMPLE((ACIN+D)*B)
      | RNDSIMPLE((ACIN+D)*B+CARRYIN)
      | RNDSIMPLE((ACIN+D)*BCIN)
      | RNDSIMPLE((ACIN+D)*BCIN+CARRYIN)
      | RNDSIMPLE((ACIN+D)+CARRYIN)
      | RNDSIMPLE((D+A))
      | RNDSIMPLE((D+A)*B)
      | RNDSIMPLE((D+A)*B+CARRYIN)
      | RNDSIMPLE((D+A)*BCIN)
      | RNDSIMPLE((D+A)*BCIN+CARRYIN)
      | RNDSIMPLE((D+A)+CARRYIN)
      | RNDSIMPLE((D+ACIN))
      | RNDSIMPLE((D+ACIN)*B)
      | RNDSIMPLE((D+ACIN)*B+CARRYIN)
      | RNDSIMPLE((D+ACIN)*BCIN)
      | RNDSIMPLE((D+ACIN)*BCIN+CARRYIN)
      | RNDSIMPLE((D+ACIN)+CARRYIN)
      | RNDSIMPLE((D-A))
      | RNDSIMPLE((D-A)*B)
      | RNDSIMPLE((D-A)*B+CARRYIN)
      | RNDSIMPLE((D-A)*BCIN)
      | RNDSIMPLE((D-A)*BCIN+CARRYIN)
      | RNDSIMPLE((D-A)+CARRYIN)
      | RNDSIMPLE((D-ACIN))
      | RNDSIMPLE((D-ACIN)*B)
      | RNDSIMPLE((D-ACIN)*B+CARRYIN)
      | RNDSIMPLE((D-ACIN)*BCIN)
      | RNDSIMPLE((D-ACIN)*BCIN+CARRYIN)
      | RNDSIMPLE((D-ACIN)+CARRYIN)
      | RNDSIMPLE(A)
      | RNDSIMPLE(A*B)
      | RNDSIMPLE(A*B+CARRYIN)
      | RNDSIMPLE(A*BCIN)
      | RNDSIMPLE(A*BCIN+CARRYIN)
      | RNDSIMPLE(A+CARRYIN)
      | RNDSIMPLE(ACIN)
      | RNDSIMPLE(ACIN*B)
      | RNDSIMPLE(ACIN*B+CARRYIN)
      | RNDSIMPLE(ACIN*BCIN)
      | RNDSIMPLE(ACIN*BCIN+CARRYIN)
      | RNDSIMPLE(ACIN+CARRYIN)
      | RNDSIMPLE(B*(A+D))
      | RNDSIMPLE(B*(A+D)+CARRYIN)
      | RNDSIMPLE(B*(ACIN+D))
      | RNDSIMPLE(B*(ACIN+D)+CARRYIN)
      | RNDSIMPLE(B*(D+A))
      | RNDSIMPLE(B*(D+A)+CARRYIN)
      | RNDSIMPLE(B*(D+ACIN))
      | RNDSIMPLE(B*(D+ACIN)+CARRYIN)
      | RNDSIMPLE(B*(D-A))
      | RNDSIMPLE(B*(D-A)+CARRYIN)
      | RNDSIMPLE(B*(D-ACIN))
      | RNDSIMPLE(B*(D-ACIN)+CARRYIN)
      | RNDSIMPLE(B*A)
      | RNDSIMPLE(B*A+CARRYIN)
      | RNDSIMPLE(B*ACIN)
      | RNDSIMPLE(B*ACIN+CARRYIN)
      | RNDSIMPLE(B*D)
      | RNDSIMPLE(B*D+CARRYIN)
      | RNDSIMPLE(BCIN*(A+D))
      | RNDSIMPLE(BCIN*(A+D)+CARRYIN)
      | RNDSIMPLE(BCIN*(ACIN+D))
      | RNDSIMPLE(BCIN*(ACIN+D)+CARRYIN)
      | RNDSIMPLE(BCIN*(D+A))
      | RNDSIMPLE(BCIN*(D+A)+CARRYIN)
      | RNDSIMPLE(BCIN*(D+ACIN))
      | RNDSIMPLE(BCIN*(D+ACIN)+CARRYIN)
      | RNDSIMPLE(BCIN*(D-A))
      | RNDSIMPLE(BCIN*(D-A)+CARRYIN)
      | RNDSIMPLE(BCIN*(D-ACIN))
      | RNDSIMPLE(BCIN*(D-ACIN)+CARRYIN)
      | RNDSIMPLE(BCIN*A)
      | RNDSIMPLE(BCIN*A+CARRYIN)
      | RNDSIMPLE(BCIN*ACIN)
      | RNDSIMPLE(BCIN*ACIN+CARRYIN)
      | RNDSIMPLE(BCIN*D)
      | RNDSIMPLE(BCIN*D+CARRYIN)
      | RNDSIMPLE(CARRYIN)
      | RNDSIMPLE(CONCAT)
      | RNDSIMPLE(CONCAT+CARRYCASCIN)
      | RNDSIMPLE(CONCAT+CARRYIN)
      | RNDSIMPLE(D)
      | RNDSIMPLE(D*B)
      | RNDSIMPLE(D*B+CARRYIN)
      | RNDSIMPLE(D*BCIN)
      | RNDSIMPLE(D*BCIN+CARRYIN)
      | RNDSIMPLE(D+CARRYIN)
      | RNDSIMPLE(P)
      | RNDSIMPLE(P+CARRYCASCIN)
      | RNDSIMPLE(P+CARRYIN)
      | RNDSIMPLE(P+CONCAT)
      | RNDSIMPLE(P+CONCAT+CARRYIN)
      | RNDSIMPLE(P+P)
      | RNDSIMPLE(P+P+CARRYIN)
      | RNDSIMPLE(P>>17)
      | RNDSIMPLE(P>>17+CARRYIN)
      | RNDSIMPLE(P>>17+CONCAT)
      | RNDSIMPLE(P>>17+CONCAT+CARRYIN)
      | RNDSIMPLE(P>>17+P)
      | RNDSIMPLE(P>>17+P+CARRYIN)
      | RNDSIMPLE(PCIN)
      | RNDSIMPLE(PCIN+CARRYIN)
      | RNDSIMPLE(PCIN+CONCAT)
      | RNDSIMPLE(PCIN+CONCAT+CARRYIN)
      | RNDSIMPLE(PCIN+P)
      | RNDSIMPLE(PCIN+P+CARRYIN)
      | RNDSIMPLE(PCIN>>17)
      | RNDSIMPLE(PCIN>>17+CARRYIN)
      | RNDSIMPLE(PCIN>>17+CONCAT)
      | RNDSIMPLE(PCIN>>17+CONCAT+CARRYIN)
      | RNDSIMPLE(PCIN>>17+P)
      | RNDSIMPLE(PCIN>>17+P+CARRYIN)
      | RNDSYM((A+D))
      | RNDSYM((A+D)*B)
      | RNDSYM((A+D)*BCIN)
      | RNDSYM((ACIN+D))
      | RNDSYM((ACIN+D)*B)
      | RNDSYM((ACIN+D)*BCIN)
      | RNDSYM((D+A))
      | RNDSYM((D+A)*B)
      | RNDSYM((D+A)*BCIN)
      | RNDSYM((D+ACIN))
      | RNDSYM((D+ACIN)*B)
      | RNDSYM((D+ACIN)*BCIN)
      | RNDSYM((D-A))
      | RNDSYM((D-A)*B)
      | RNDSYM((D-A)*BCIN)
      | RNDSYM((D-ACIN))
      | RNDSYM((D-ACIN)*B)
      | RNDSYM((D-ACIN)*BCIN)
      | RNDSYM(A)
      | RNDSYM(A*B)
      | RNDSYM(A*BCIN)
      | RNDSYM(ACIN)
      | RNDSYM(ACIN*B)
      | RNDSYM(ACIN*BCIN)
      | RNDSYM(B*(A+D))
      | RNDSYM(B*(ACIN+D))
      | RNDSYM(B*(D+A))
      | RNDSYM(B*(D+ACIN))
      | RNDSYM(B*(D-A))
      | RNDSYM(B*(D-ACIN))
      | RNDSYM(B*A)
      | RNDSYM(B*ACIN)
      | RNDSYM(B*D)
      | RNDSYM(BCIN*(A+D))
      | RNDSYM(BCIN*(ACIN+D))
      | RNDSYM(BCIN*(D+A))
      | RNDSYM(BCIN*(D+ACIN))
      | RNDSYM(BCIN*(D-A))
      | RNDSYM(BCIN*(D-ACIN))
      | RNDSYM(BCIN*A)
      | RNDSYM(BCIN*ACIN)
      | RNDSYM(BCIN*D)
      | RNDSYM(D)
      | RNDSYM(D*B)
      | RNDSYM(D*BCIN)
      | RNDSYM(P)
      | RNDSYM(PCIN)'
      dspimage=|
      | <!DOCTYPE HTML PUBLIC "-//W3C//DTD HTML 4.0//EN" "http://www.w3.org/TR/REC-html40/strict.dtd">
      | <html><head><meta name="qrichtext" content="1" /><style type="text/css">
      | p, li { white-space: pre-wrap; }
      | </style></head><body style=" font-family:'Sans Serif'; font-size:12pt; font-weight:400; font-style:normal;">
      | <p style=" margin-top:0px; margin-bottom:0px; margin-left:0px; margin-right:0px; -qt-block-indent:0; text-indent:0px;"><img src="/opt/Xilinx/14.7/ISE_DS/ISE/sysgen/data/images/xbip_dsp48_macro_v2_1_regimag.png" /></p></body></html>
      settings: infoedit=<html>Valid operands: CONCAT, P, C, PCIN, P>>17, PCIN>>17, CARRYIN, CARRYCASCIN, ACIN, A, BCIN,B<br><br>Valid operators: +, -, *, ()<br><br>Valid functions: RNDSIMPLE, RNDSYM<br><br>Instructions are case insensitive and tolerate spaces.</html>
  Register0 : xbsIndex_r4/Register  init=0  rst=off  en=off  dbl_ovrd=off  block_type=register
  Register1 : xbsIndex_r4/Register  init=0  rst=off  en=off  dbl_ovrd=off  block_type=register
  Register3 : xbsIndex_r4/Register  init=0  rst=off  en=off  dbl_ovrd=off  block_type=register
  sym_out : Outport
  sum_out : Outport  Port=2
  wires:
  Register3/1 -> DSP48 Macro_0/3
  Register0/1 -> sym_out/1
  Register1/1 -> DSP48 Macro_0/1, Register0/1
  samp_in/1 -> Register1/1
  DSP48 Macro_0/1 -> sum_out/1
  Constant0/1 -> DSP48 Macro_0/2
  sum_in/1 -> Register3/1
